simulink model "H175_PANKL_V1a"  (R2023a)
settings: Solver=ode15s  StartTime=0.0  StopTime=22136  RelTol=1e-3  AbsTol=1e-3
PreLoadFcn:
  | omega_TLU = [1000, 1500, 2000, 2500, 3000, 3500];
  | beta_TLU = linspace(0,1,7);
  | 
  | mdot_TLU = [0.1377    0.1304    0.1187    0.1029    0.0854    0.0658    0.0437
  |     0.2310    0.2183    0.1978    0.1688    0.1400    0.1118    0.0750
  |     0.3298    0.3208    0.2987    0.2677    0.2256    0.1774    0.1194
  |     0.4520    0.4260    0.3825    0.3308    0.2745    0.2227    0.1655
  |     0.5542    0.5353    0.4781    0.4230    0.3477    0.2897    0.2211
  |     0.6197    0.5805    0.5198    0.4516    0.3971    0.3555    0.2825];
  | 
  | eta_TLU = [0.7905    0.8025    0.7998    0.7972    0.7932    0.7882    0.7827
  |     0.7993    0.8239    0.8350    0.8379    0.8197    0.8000    0.7809
  |     0.8011    0.8374    0.8632    0.8827    0.8749    0.8394    0.7948
  |     0.8072    0.8520    0.8814    0.9000    0.8676    0.8356    0.7971
  |     0.8076    0.8271    0.8608    0.8766    0.8529    0.8329    0.7992
  |     0.7949    0.8131    0.8296    0.8243    0.8170    0.8085    0.7972];
  | 
  | pr_TLU = [1.0912    1.1795    1.2293    1.2662    1.2928    1.3108    1.3151
  |     1.1484    1.3081    1.3958    1.4707    1.5136    1.5380    1.5456
  |     1.2830    1.4539    1.5943    1.7042    1.7973    1.8582    1.8799
  |     1.5180    1.8034    1.9693    2.0899    2.1662    2.2027    2.2182
  |     1.8359    2.0956    2.3359    2.4668    2.5687    2.6106    2.6224
  |     2.3061    2.6623    2.8585    2.9837    3.0443    3.0714    3.0869];
values from neighbouring files (symbols this model uses):
  P64_omega_TLU = [44762 68636 92509 110414 125335 137271 146224]    [All_Properties.mat]    (also in PANKL_CMP.mat = [44762 68636 92509 110414 125335 137271 146224 155176.0695 1)
libraries: fl_lib x101, nesl_utility x76, SimscapeFluids_lib x5, slpidlib x3
(part 1 of 4)
CloseFcn:
  | clear tout simlogCompressorMap
  | clear omega_TLU
  | clear beta_TLU
  | clear mdot_TLU
  | clear pr_TLU
  | clear eta_TLU
Description:
  | Compressor Map
settings Model: Creator=The MathWorks, Inc.  LastModifiedBy=H2FADMIN
settings SolverCC: AutoScaleAbsTol=off  MaxConsecutiveMinStep=50  ZeroCrossAlgorithm=Adaptive  AlgebraicLoopSolver=TrustRegion  MaxZcPerStep=1
settings DataIOCC: ReturnWorkspaceOutputs=off
settings OptimizationCC: ReuseModelBlockBuffer=off
settings DebuggingCC: AlgebraicLoopMsg=none  IgnoredZcDiagnostic=none  UnconnectedInputMsg=warning  UnconnectedOutputMsg=warning  UnconnectedLineMsg=warning  SymbolicDimsDataTypeCodeGenerationDiagnostic=none
settings ModelReferenceCC: EnableRefExpFcnMdlSchedulingChecks=on
settings SFSimCC: CustomCodeUndefinedFunction=UseInterfaceOnly
settings RTWCC: DLArmComputeVersion=19.05
settings SimscapeCC: SimscapeLogType=all  SimscapeLogSimulationStatistics=on  SimscapeLogName=simlog_H175_PANKL_V1b  SimscapeLogDataHistory=10000

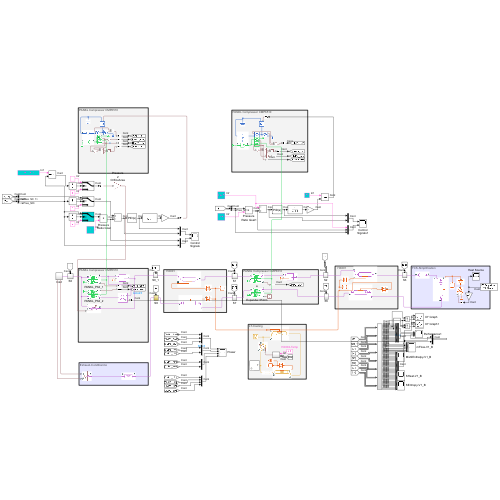
[thumbnail: Simulink's stored preview of the top-level diagram]
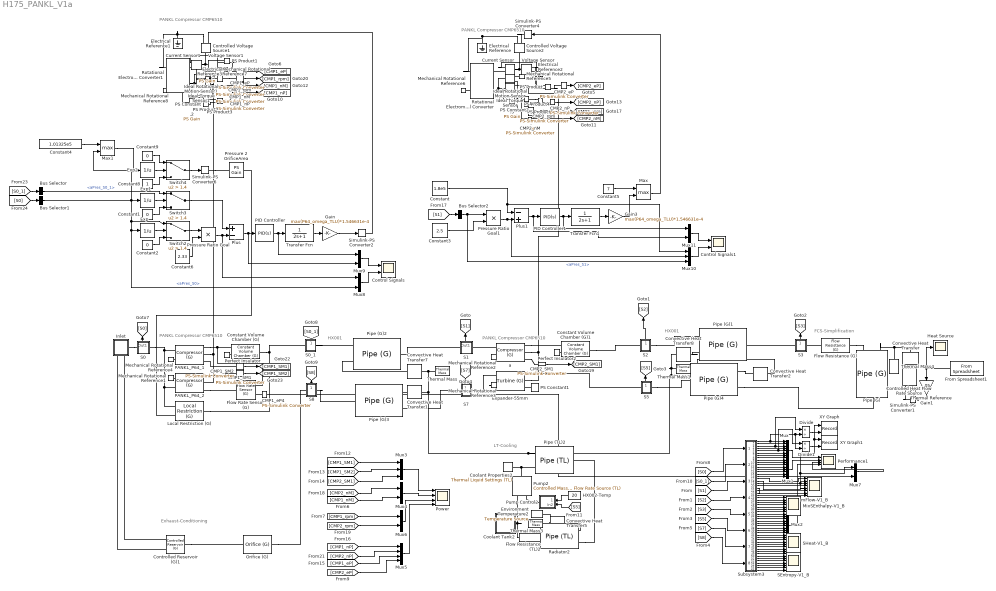
== system H175_PANKL_V1a ==
  note: PANKL Compressor CMP6510
  note: FCS-Simplification
  note: Exhaust-Conditioning
  note: PANKL Compressor CMP6510
  note: HX001
  note: HX001
  note: LT-Cooling
  note: PANKL Compressor CMP6510
  note: PANKL Compressor CMP6510
  . : fl_lib/Physical Signals/Functions/PS Gain  gain=1/(0.1047198*1000)
  .2 : fl_lib/Physical Signals/Functions/PS Gain  gain=1/(0.1047198*60)
  .3 : fl_lib/Physical Signals/Functions/PS Gain  gain=1/(0.1047198*60)
  .4 : fl_lib/Physical Signals/Functions/PS Gain  gain=1/(0.1047198*1000)
  Bus Selector : BusSelector  OutputSignals=aPres_S0_1
  Bus Selector1 : BusSelector  OutputSignals=aPres_S0
  Bus Selector2 : BusSelector  OutputSignals=aPres_S1
  CMP1_SM1 : nesl_utility/PS-Simulink Converter  PhysicalDomain=network_engine_domain  SubClassName=ps_output  LeftPortType=input  RightPortType=output  PseudoPeriodic=off  Frequencies=[]  VectorFormat=inherit  Unit=inherit  AffineConversion=off
  CMP1_SM2 : nesl_utility/PS-Simulink Converter  PhysicalDomain=network_engine_domain  SubClassName=ps_output  LeftPortType=input  RightPortType=output  PseudoPeriodic=off  Frequencies=[]  VectorFormat=inherit  Unit=inherit  AffineConversion=off
  CMP1_eP : nesl_utility/PS-Simulink Converter  PhysicalDomain=network_engine_domain  SubClassName=ps_output  LeftPortType=input  RightPortType=output  PseudoPeriodic=off  Frequencies=[]  VectorFormat=inherit  Unit=inherit  AffineConversion=off
  CMP1_eP4 : nesl_utility/PS-Simulink Converter  PhysicalDomain=network_engine_domain  SubClassName=ps_output  LeftPortType=input  RightPortType=output  PseudoPeriodic=off  Frequencies=[]  VectorFormat=inherit  Unit=inherit  AffineConversion=off
  CMP1_nM : nesl_utility/PS-Simulink Converter  PhysicalDomain=network_engine_domain  SubClassName=ps_output  LeftPortType=input  RightPortType=output  PseudoPeriodic=off  Frequencies=[]  VectorFormat=1-D array  Unit=inherit  AffineConversion=off
  CMP1_nP : nesl_utility/PS-Simulink Converter  PhysicalDomain=network_engine_domain  SubClassName=ps_output  LeftPortType=input  RightPortType=output  PseudoPeriodic=off  Frequencies=[]  VectorFormat=inherit  Unit=inherit  AffineConversion=off
  CMP1_rpm : nesl_utility/PS-Simulink Converter  PhysicalDomain=network_engine_domain  SubClassName=ps_output  LeftPortType=input  RightPortType=output  PseudoPeriodic=off  Frequencies=[]  VectorFormat=inherit  Unit=inherit  AffineConversion=off
  CMP2_SM1 : nesl_utility/PS-Simulink Converter  PhysicalDomain=network_engine_domain  SubClassName=ps_output  LeftPortType=input  RightPortType=output  PseudoPeriodic=off  Frequencies=[]  VectorFormat=inherit  Unit=inherit  AffineConversion=off
  CMP2_eP : nesl_utility/PS-Simulink Converter  PhysicalDomain=network_engine_domain  SubClassName=ps_output  LeftPortType=input  RightPortType=output  PseudoPeriodic=off  Frequencies=[]  VectorFormat=inherit  Unit=inherit  AffineConversion=off
  CMP2_nM : nesl_utility/PS-Simulink Converter  PhysicalDomain=network_engine_domain  SubClassName=ps_output  LeftPortType=input  RightPortType=output  PseudoPeriodic=off  Frequencies=[]  VectorFormat=1-D array  Unit=inherit  AffineConversion=off
  CMP2_nP : nesl_utility/PS-Simulink Converter  PhysicalDomain=network_engine_domain  SubClassName=ps_output  LeftPortType=input  RightPortType=output  PseudoPeriodic=off  Frequencies=[]  VectorFormat=inherit  Unit=inherit  AffineConversion=off
  CMP2_rpm : nesl_utility/PS-Simulink Converter  PhysicalDomain=network_engine_domain  SubClassName=ps_output  LeftPortType=input  RightPortType=output  PseudoPeriodic=off  Frequencies=[]  VectorFormat=inherit  Unit=inherit  AffineConversion=off
  Constant : Constant  Value=1.8e5
  Constant Volume Chamber (G) : fl_lib/Gas/Elements/Constant Volume Chamber (G)  volume=1 l  num_ports=foundation.enum.num_ports.two  area_A=0.1 m^2  area_B=0.005 m^2  area_C=0.01 m^2  area_D=0.01 m^2  p_I_specify=off  p_I_priority=High  p_I=0.101325 MPa  p_I_nominal_specify=off  p_I_nominal_unit=MPa  p_I_nominal_value=1  T_I_specify=off  T_I_priority=High  T_I=293.15 K  T_I_nominal_specify=off  T_I_nominal_unit=K  T_I_nominal_value=1  rho_I_specify=off  rho_I_priority=None  rho_I=1.2 kg/m^3  rho_I_nominal_specify=off  rho_I_nominal_unit=kg/m^3  rho_I_nominal_value=1
      settings: InternalSimscapePortConfiguration="{\"Bottom\":[],\"Left\":[{\"id\":\"A\",\"label\":\"A\",\"type\":\"foundation.gas.gas\"},{\"id\":\"H\",\"label\":\"H\",\"type\":\"foundation.thermal.thermal\"}],\"Right\":[{\"id\":\"B\",\"label\":\"B\",\"type\":\"foundation.gas.gas\"}],\"Top\":[]}"
  Constant Volume Chamber (G)1 : fl_lib/Gas/Elements/Constant Volume Chamber (G)  volume=1 l  num_ports=foundation.enum.num_ports.two  area_A=0.1 m^2  area_B=0.005 m^2  area_C=0.01 m^2  area_D=0.01 m^2  p_I_specify=off  p_I_priority=High  p_I=0.101325 MPa  p_I_nominal_specify=off  p_I_nominal_unit=MPa  p_I_nominal_value=1  T_I_specify=off  T_I_priority=High  T_I=293.15 K  T_I_nominal_specify=off  T_I_nominal_unit=K  T_I_nominal_value=1  rho_I_specify=off  rho_I_priority=None  rho_I=1.2 kg/m^3  rho_I_nominal_specify=off  rho_I_nominal_unit=kg/m^3  rho_I_nominal_value=1
      settings: InternalSimscapePortConfiguration="{\"Bottom\":[],\"Left\":[{\"id\":\"A\",\"label\":\"A\",\"type\":\"foundation.gas.gas\"},{\"id\":\"H\",\"label\":\"H\",\"type\":\"foundation.thermal.thermal\"}],\"Right\":[{\"id\":\"B\",\"label\":\"B\",\"type\":\"foundation.gas.gas\"}],\"Top\":[]}"
  Constant1 : Constant  Value=0
  Constant2 : Constant  Value=0
  Constant3 : Constant  Value=2.5
  Constant4 : Constant  Value=1.01325e5
  Constant5 : Constant  Value=7
  Constant6 : Constant  Value=2.33
  Constant8 : Constant
  Constant9 : Constant  Value=0
  Control Signals : Scope  NumInputPorts=2
  Control Signals1 : Scope  NumInputPorts=2
  Controlled Heat Flow Rate Source : fl_lib/Thermal/Thermal Sources/Controlled Heat Flow Rate Source
  Controlled Reservoir (G)1 : fl_lib/Gas/Elements/Controlled Reservoir (G)  area_A=0.002 m^2
      settings: InternalSimscapePortConfiguration="{\"Bottom\":[],\"Left\":[{\"id\":\"A\",\"label\":\"A\",\"type\":\"foundation.gas.gas\"}],\"Right\":[{\"id\":\"T_in\",\"label\":\"T\",\"type\":\"input\"},{\"id\":\"p_in\",\"label\":\"P\",\"type\":\"input\"}],\"Top\":[]}"
  Controlled Voltage Source1 : fl_lib/Electrical/Electrical Sources/Controlled Voltage Source
  Controlled Voltage Source2 : fl_lib/Electrical/Electrical Sources/Controlled Voltage Source
  Convective Heat Transfer : fl_lib/Thermal/Thermal Elements/Convective Heat Transfer  thermal_type=foundation.enum.constant_variable.constant  area=.25 m^2  heat_tr_coeff=200 W/(K*m^2)  min_heat_tr_coeff=1e-3 W/(K*m^2)  T_specify=on  T_priority=None  T=10 K  T_nominal_specify=off  T_nominal_unit=K  T_nominal_value=1  Q_specify=off  Q_priority=None  Q=0 W  Q_nominal_specify=off  Q_nominal_unit=W  Q_nominal_value=1
  Convective Heat Transfer1 : fl_lib/Thermal/Thermal Elements/Convective Heat Transfer  thermal_type=foundation.enum.constant_variable.constant  area=100 cm^2  heat_tr_coeff=1000 W/(m^2 * K)  min_heat_tr_coeff=1e-3 W/(K*m^2)  T_specify=off  T_priority=None  T=0 K  T_nominal_specify=off  T_nominal_unit=K  T_nominal_value=1  Q_specify=off  Q_priority=None  Q=0 W  Q_nominal_specify=off  Q_nominal_unit=W  Q_nominal_value=1
  Convective Heat Transfer2 : fl_lib/Thermal/Thermal Elements/Convective Heat Transfer  thermal_type=foundation.enum.constant_variable.constant  area=100 cm^2  heat_tr_coeff=1000 W/(m^2 * K)  min_heat_tr_coeff=1e-3 W/(K*m^2)  T_specify=off  T_priority=None  T=0 K  T_nominal_specify=off  T_nominal_unit=K  T_nominal_value=1  Q_specify=off  Q_priority=None  Q=0 W  Q_nominal_specify=off  Q_nominal_unit=W  Q_nominal_value=1
  Convective Heat Transfer5 : fl_lib/Thermal/Thermal Elements/Convective Heat Transfer  thermal_type=foundation.enum.constant_variable.constant  area=5 m^2  heat_tr_coeff=300 W/(m^2 * K)  min_heat_tr_coeff=1e-3 W/(K*m^2)  T_specify=off  T_priority=None  T=0 K  T_nominal_specify=off  T_nominal_unit=K  T_nominal_value=1  Q_specify=off  Q_priority=None  Q=0 W  Q_nominal_specify=off  Q_nominal_unit=W  Q_nominal_value=1
  Convective Heat Transfer7 : fl_lib/Thermal/Thermal Elements/Convective Heat Transfer  thermal_type=foundation.enum.constant_variable.constant  area=100 cm^2  heat_tr_coeff=50000 W/(m^2 * K)  min_heat_tr_coeff=1e-3 W/(K*m^2)  T_specify=off  T_priority=None  T=0 K  T_nominal_specify=off  T_nominal_unit=K  T_nominal_value=1  Q_specify=off  Q_priority=None  Q=0 W  Q_nominal_specify=off  Q_nominal_unit=W  Q_nominal_value=1
  Convective Heat Transfer8 : fl_lib/Thermal/Thermal Elements/Convective Heat Transfer  thermal_type=foundation.enum.constant_variable.constant  area=100 cm^2  heat_tr_coeff=100000 W/(m^2 * K)  min_heat_tr_coeff=1e-3 W/(K*m^2)  T_specify=off  T_priority=None  T=0 K  T_nominal_specify=off  T_nominal_unit=K  T_nominal_value=1  Q_specify=off  Q_priority=None  Q=0 W  Q_nominal_specify=off  Q_nominal_unit=W  Q_nominal_value=1
  Coolant Properties2 : fl_lib/Thermal Liquid/Utilities/Thermal Liquid Settings (TL)  table_dimensions=foundation.enum.table_dimensions_TL.two_dimensional  T_TLU=[273.1600 : 10 : 373.16]' K  p_TLU=[0.01, 0.1, 5 : 5 : 50] MPa  p_atm=0.101325 MPa  pT_region_flag=foundation.enum.pT_region_TL.min_max  T_min=273.16 K  T_max=373.16 K  p_min=0.05 MPa  p_max=50 MPa  T_min_1D=273.16 K  T_max_1D=363.16 K  p_min_1D=0.05 MPa  p_max_1D=50 MPa  pT_validity_TLU=[1, 1, 1, 1, 1, 1, 1, 1, 1, 1, 1, 1; 1, 1, 1, 1, 1, 1, 1, 1, 1, 1, 1, 1; 1, 1, 1, 1, 1, 1, 1, 1, 1, 1, 1, 1; 1, 1, 1, 1, 1, 1, 1, 1, 1, 1, 1, 1; 1, 1, 1, 1, 1, 1, 1, 1, 1, 1, 1, 1; 0, 1, 1, 1, 1, 1, 1, 1, 1, 1, 1, 1; 0, 1, 1, 1, 1, 1, 1, 1, 1, 1, 1, 1; 0, 1, 1, 1, 1, 1, 1, 1, 1, 1, 1, 1; 0, 1, 1, 1, 1, 1, 1, 1, 1, 1, 1, 1; 0, 1, 1, 1, 1, 1, 1, 1, 1, 1, 1, 1; 0, 0, 1, 1, 1, 1, 1, 1, 1, 1, 1, 1]  properties_range_check=simscape.enum.assert.action.error  rho_parameterization_2D=foundation.enum.rho_parameterization_2D.rho_beta_alpha  rho_parameterization_1D=foundation.enum.rho_parameterization_1D.rho_vector  rho_TLU=[999.7973, 999.8431, 1002.3216, 1004.8218, 1007.293, 1009.7358, 1012.1506, 1014.5379, 1016.8979, 1019.2311, 1021.538, 1023.8188; 999.6579, 999.7009, 1002.0303, 1004.382, 1006.7084, 1009.0101, 1011.2874, 1013.5407, 1015.7703, 1017.9766, 1020.1599, 1022.3206; 998.1632, 998.2045, 1000.4375, 1002.6924, 1004.9239, 1007.1324, 1009.3183, 1011.4819, 1013.6236, 1015.7438, 1017.8428, 1019.921; 995.6057, 995.6458, 997.81864, 1000.0128, 1002.1841, 1004.3332, 1006.4603, 1008.566, 1010.6505, 1012.7144, 1014.758, 1016.7815; 992.1724, 992.2119, 994.35133, 996.5113, 998.6484, 1000.7633, 1002.8563, 1004.928, 1006.9788, 1009.009, 1011.0192, 1013.0097; 988.02, 988.0299, 990.15684, 992.3035, 994.4268, 996.5273, 998.6056, 1000.6622, 1002.6976, 1004.7123, 1006.7067, 1008.6813; 983.18, 983.1901, 985.3217, 987.4721, 989.5983, 991.7008, 993.7803, 995.8374, 997.8726, 999.8864, 1001.8795, 1003.8522; 977.75, 977.7583, 979.9094, 982.0783, 984.2216, 986.34, 988.4343, 990.505, 992.5529, 994.5786, 996.5825, 998.5654; 971.77, 971.7836, 973.96734, 976.1678, 978.3409, 980.4876, 982.6087, 984.7049, 986.7768, 988.8254, 990.8511, 992.8545; 965.26, 965.3023, 967.53107, 969.7753, 971.9901, 974.1764, 976.3354, 978.4676, 980.5741, 982.6556, 984.7129, 986.7465; 958.62, 958.6315, 960.627, 962.9267, 965.1944, 967.4314, 969.6387, 971.8173, 973.9681, 976.0921, 978.19, 980.2628] kg/m^3  beta_TLU=[1.9649, 1.9654, 1.9929, 2.0213, 2.0499, 2.0787, 2.1078, 2.1372, 2.1668, 2.1966, 2.2268, 2.2572; 2.0913, 2.0918, 2.1191, 2.1471, 2.1752, 2.2036, 2.2322, 2.261, 2.2899, 2.3191, 2.3485, 2.3781; 2.1786, 2.1791, 2.2067, 2.235, 2.2634, 2.2919, 2.3206, 2.3494, 2.3784, 2.4075, 2.4367, 2.4661; 2.2332, 2.2337, 2.2619, 2.2908, 2.3197, 2.3487, 2.3778, 2.407, 2.4363, 2.4657, 2.4951, 2.5246; 2.26, 2.2605, 2.2895, 2.3191, 2.3487, 2.3784, 2.4081, 2.4378, 2.4675, 2.4973, 2.5272, 2.5571; 2.2638, 2.2638, 2.2936, 2.324, 2.3544, 2.3848, 2.4151, 2.4455, 2.4758, 2.5062, 2.5365, 2.5669; 2.2472, 2.2472, 2.2779, 2.3092, 2.3403, 2.3715, 2.4025, 2.4336, 2.4646, 2.4955, 2.5264, 2.5573; 2.214, 2.214, 2.2455, 2.2776, 2.3096, 2.3415, 2.3733, 2.405, 2.4367, 2.4683, 2.4998, 2.5313; 2.1668, 2.1668, 2.1992, 2.2321, 2.2649, 2.2976, 2.3301, 2.3626, 2.3949, 2.4272, 2.4593, 2.4914; 2.1081, 2.1081, 2.1413, 2.175, 2.2086, 2.2421, 2.2754, 2.3085, 2.3415, 2.3744, 2.4072, 2.4399; 2.0494, 2.0494, 2.0739, 2.1084, 2.1428, 2.177, 2.211, 2.2449, 2.2786, 2.3121, 2.3455, 2.3788] GPa  alpha_TLU=1e-4 * [-.679, -.676, -.49, -.307, -.13, .041, .206, .365, .519, .668, .811, .949; .878, .881, .998, 1.114, 1.227, 1.337, 1.445, 1.549, 1.651, 1.75, 1.846, 1.939; 2.068, 2.069, 2.141, 2.213, 2.283, 2.352, 2.42, 2.486, 2.551, 2.614, 2.676, 2.736; 3.034, 3.035, 3.074, 3.113, 3.152, 3.191, 3.229, 3.267, 3.305, 3.341, 3.377, 3.413; 3.855, 3.856, 3.87, 3.884, 3.899, 3.914, 3.93, 3.946, 3.961, 3.977, 3.993, 4.009; 4.578, 4.578, 4.572, 4.566, 4.562, 4.558, 4.555, 4.552, 4.55, 4.549, 4.548, 4.547; 5.233, 5.233, 5.209, 5.186, 5.165, 5.144, 5.125, 5.107, 5.09, 5.074, 5.059, 5.045; 5.84, 5.84, 5.801, 5.762, 5.725, 5.691, 5.657, 5.625, 5.595, 5.566, 5.538, 5.512; 6.414, 6.414, 6.36, 6.307, 6.256, 6.208, 6.161, 6.117, 6.074, 6.033, 5.994, 5.956; 6.967, 6.967, 6.898, 6.831, 6.766, 6.705, 6.646, 6.589, 6.535, 6.482, 6.432, 6.384; 7.519, 7.519, 7.423, 7.342, 7.264, 7.189, 7.118, 7.049, 6.983, 6.92, 6.859, 6.8] 1/K  rho_TLU_2=[999.7973, 999.8431, 1002.3216, 1004.8218, 1007.293, 1009.7358, 1012.1506, 1014.5379, 1016.8979, 1019.2311, 1021.538, 1023.8188; 999.6579, 999.7009, 1002.0303, 1004.382, 1006.7084, 1009.0101, 1011.2874, 1013.5407, 1015.7703, 1017.9766, 1020.1599, 1022.3206; 998.1632, 998.2045, 1000.4375, 1002.6924, 1004.9239, 1007.1324, 1009.3183, 1011.4819, 1013.6236, 1015.7438, 1017.8428, 1019.921; 995.6057, 995.6458, 997.81864, 1000.0128, 1002.1841, 1004.3332, 1006.4603, 1008.566, 1010.6505, 1012.7144, 1014.758, 1016.7815; 992.1724, 992.2119, 994.35133, 996.5113, 998.6484, 1000.7633, 1002.8563, 1004.928, 1006.9788, 1009.009, 1011.0192, 1013.0097; 988.02, 988.0299, 990.15684, 992.3035, 994.4268, 996.5273, 998.6056, 1000.6622, 1002.6976, 1004.7123, 1006.7067, 1008.6813; 983.18, 983.1901, 985.3217, 987.4721, 989.5983, 991.7008, 993.7803, 995.8374, 997.8726, 999.8864, 1001.8795, 1003.8522; 977.75, 977.7583, 979.9094, 982.0783, 984.2216, 986.34, 988.4343, 990.505, 992.5529, 994.5786, 996.5825, 998.5654; 971.77, 971.7836, 973.96734, 976.1678, 978.3409, 980.4876, 982.6087, 984.7049, 986.7768, 988.8254, 990.8511, 992.8545; 965.26, 965.3023, 967.53107, 969.7753, 971.9901, 974.1764, 976.3354, 978.4676, 980.5741, 982.6556, 984.7129, 986.7465; 958.62, 958.6315, 960.627, 962.9267, 965.1944, 967.4314, 969.6387, 971.8173, 973.9681, 976.0921, 978.19, 980.2628] kg/m^3  rho_ref_3=998.21 kg/m^3  T_ref_3=293.16 K  p_ref_3=0.101325 MPa  beta_const_3=2.1791 GPa  alpha_const_3=2.0691e-4 1/K  rho_TLU_4=[999.84; 999.7; 998.2; 995.65; 992.21; 988.03; 983.19; 977.76; 971.78; 965.3; 958.8] kg/m^3  beta_const_4=2.1791 GPa  p_ref_4=0.101325 MPa  rho_ref_5=998.21 kg/m^3  T_ref_5=293.16 K  p_ref_5=0.101325 MPa  beta_const_5=2.1791 GPa  alpha_const_5=2.0691e-4 1/K  u_parameterization_2D=foundation.enum.u_parameterization_2D.u_cp  u_parameterization_1D=foundation.enum.u_parameterization_1D.u  u_TLU=[.0002, .0018, .086, .1588, .219, .267, .3034, .3288, .3436, .3483, .3435, .3294; 42.062, 42.06, 41.935, 41.804, 41.668, 41.527, 41.382, 41.233, 41.081, 40.924, 40.763, 40.599; 83.953, 83.948, 83.651, 83.349, 83.049, 82.749, 82.451, 82.153, 81.856, 81.56, 81.265, 80.971; 125.77, 125.76, 125.31, 124.86, 124.41, 123.97, 123.53, 123.1, 122.68, 122.25, 121.84, 121.42; 167.57, 167.56, 166.96, 166.37, 165.79, 165.21, 164.65, 164.09, 163.54, 163, 162.46, 161.94; 209.36, 209.36, 208.63, 207.9, 207.19, 206.48, 205.79, 205.11, 204.45, 203.79, 203.14, 202.5; 251.19, 251.19, 250.33, 249.47, 248.62, 247.79, 246.98, 246.18, 245.39, 244.62, 243.86, 243.12; 293.06, 293.06, 292.07, 291.07, 290.1, 289.14, 288.2, 287.28, 286.38, 285.49, 284.62, 283.77; 334.99, 334.99, 333.86, 332.73, 331.63, 330.54, 329.48, 328.44, 327.41, 326.41, 325.43, 324.46; 377, 377, 375.73, 374.46, 373.22, 372, 370.81, 369.64, 368.5, 367.38, 366.27, 365.19; 419.01, 419.01, 417.69, 416.27, 414.89, 413.54, 412.21, 410.91, 409.64, 408.4, 407.17, 405.98] kJ/kg  cp_TLU=[4.2199, 4.2194, 4.1957, 4.1726, 4.1508, 4.13, 4.1103, 4.0916, 4.0738, 4.0569, 4.0408, 4.0254; 4.1955, 4.1951, 4.1769, 4.1592, 4.1422, 4.1259, 4.1103, 4.0954, 4.0812, 4.0676, 4.0545, 4.0421; 4.1843, 4.184, 4.169, 4.1543, 4.1401, 4.1264, 4.1133, 4.1007, 4.0885, 4.0768, 4.0656, 4.0548; 4.1801, 4.1798, 4.1667, 4.1538, 4.1413, 4.1293, 4.1177, 4.1064, 4.0956, 4.0851, 4.075, 4.0653; 4.1796, 4.1794, 4.1675, 4.1558, 4.1444, 4.1334, 4.1227, 4.1123, 4.1023, 4.0926, 4.0832, 4.0741; 4.1813, 4.1813, 4.1702, 4.1592, 4.1484, 4.138, 4.1279, 4.1181, 4.1086, 4.0993, 4.0903, 4.0816; 4.185, 4.185, 4.1742, 4.1636, 4.1532, 4.1432, 4.1334, 4.1239, 4.1146, 4.1056, 4.0969, 4.0884; 4.1901, 4.1901, 4.1795, 4.169, 4.1588, 4.1489, 4.1393, 4.1299, 4.1207, 4.1118, 4.1032, 4.0947; 4.1968, 4.1968, 4.1862, 4.1757, 4.1655, 4.1555, 4.1458, 4.1364, 4.1273, 4.1183, 4.1096, 4.1012; 4.2052, 4.2052, 4.1944, 4.1837, 4.1733, 4.1632, 4.1534, 4.1438, 4.1345, 4.1255, 4.1166, 4.108; 4.2136, 4.2136, 4.2045, 4.1935, 4.1828, 4.1724, 4.1623, 4.1524, 4.1429, 4.1335, 4.1245, 4.1157] kJ/kg/K  u_TLU_2=[.0002, .0018, .086, .1588, .219, .267, .3034, .3288, .3436, .3483, .3435, .3294; 42.062, 42.06, 41.935, 41.804, 41.668, 41.527, 41.382, 41.233, 41.081, 40.924, 40.763, 40.599; 83.953, 83.948, 83.651, 83.349, 83.049, 82.749, 82.451, 82.153, 81.856, 81.56, 81.265, 80.971; 125.77, 125.76, 125.31, 124.86, 124.41, 123.97, 123.53, 123.1, 122.68, 122.25, 121.84, 121.42; 167.57, 167.56, 166.96, 166.37, 165.79, 165.21, 164.65, 164.09, 163.54, 163, 162.46, 161.94; 209.36, 209.36, 208.63, 207.9, 207.19, 206.48, 205.79, 205.11, 204.45, 203.79, 203.14, 202.5; 251.19, 251.19, 250.33, 249.47, 248.62, 247.79, 246.98, 246.18, 245.39, 244.62, 243.86, 243.12; 293.06, 293.06, 292.07, 291.07, 290.1, 289.14, 288.2, 287.28, 286.38, 285.49, 284.62, 283.77; 334.99, 334.99, 333.86, 332.73, 331.63, 330.54, 329.48, 328.44, 327.41, 326.41, 325.43, 324.46; 377, 377, 375.73, 374.46, 373.22, 372, 370.81, 369.64, 368.5, 367.38, 366.27, 365.19; 419.01, 419.01, 417.69, 416.27, 414.89, 413.54, 412.21, 410.91, 409.64, 408.4, 407.17, 405.98] kJ/kg  cp_TLU_3=[4.2199, 4.2194, 4.1957, 4.1726, 4.1508, 4.13, 4.1103, 4.0916, 4.0738, 4.0569, 4.0408, 4.0254; 4.1955, 4.1951, 4.1769, 4.1592, 4.1422, 4.1259, 4.1103, 4.0954, 4.0812, 4.0676, 4.0545, 4.0421; 4.1843, 4.184, 4.169, 4.1543, 4.1401, 4.1264, 4.1133, 4.1007, 4.0885, 4.0768, 4.0656, 4.0548; 4.1801, 4.1798, 4.1667, 4.1538, 4.1413, 4.1293, 4.1177, 4.1064, 4.0956, 4.0851, 4.075, 4.0653; 4.1796, 4.1794, 4.1675, 4.1558, 4.1444, 4.1334, 4.1227, 4.1123, 4.1023, 4.0926, 4.0832, 4.0741; 4.1813, 4.1813, 4.1702, 4.1592, 4.1484, 4.138, 4.1279, 4.1181, 4.1086, 4.0993, 4.0903, 4.0816; 4.185, 4.185, 4.1742, 4.1636, 4.1532, 4.1432, 4.1334, 4.1239, 4.1146, 4.1056, 4.0969, 4.0884; 4.1901, 4.1901, 4.1795, 4.169, 4.1588, 4.1489, 4.1393, 4.1299, 4.1207, 4.1118, 4.1032, 4.0947; 4.1968, 4.1968, 4.1862, 4.1757, 4.1655, 4.1555, 4.1458, 4.1364, 4.1273, 4.1183, 4.1096, 4.1012; 4.2052, 4.2052, 4.1944, 4.1837, 4.1733, 4.1632, 4.1534, 4.1438, 4.1345, 4.1255, 4.1166, 4.108; 4.2136, 4.2136, 4.2045, 4.1935, 4.1828, 4.1724, 4.1623, 4.1524, 4.1429, 4.1335, 4.1245, 4.1157] kJ/kg/K  u_TLU_4=[.0018; 42.06; 83.948; 125.76; 167.56; 209.36; 251.19; 293.06; 334.99; 377; 418.01] kJ/kg  cp_TLU_5=[4.2199; 4.1955; 4.1843; 4.1801; 4.1796; 4.1813; 4.185; 4.1901; 4.1968; 4.2052; 4.2136] kJ/kg/K  nu_TLU=[1.7917, 1.7914, 1.7763, 1.7615, 1.7473, 1.7338, 1.7208, 1.7085, 1.6967, 1.6854, 1.6747, 1.6645; 1.3061, 1.3059, 1.2986, 1.2914, 1.2845, 1.2779, 1.2716, 1.2656, 1.2598, 1.2543, 1.2491, 1.2441; 1.0032, 1.0032, .9995, .9959, .9924, .9891, .9859, .9829, .9801, .9774, .9748, .9724; .8006, .8005, .7987, .797, .7953, .7937, .7922, .7908, .7894, .7881, .787, .7859; .6577, .6577, .657, .6562, .6555, .6548, .6543, .6537, .6532, .6528, .6523, .652; .553, .553, .5529, .5527, .5526, .5525, .5524, .5524, .5524, .5524, .5524, .5525; .4739, .4739, .4741, .4743, .4745, .4747, .475, .4753, .4755, .4758, .4762, .4765; .4127, .4127, .4131, .4135, .4139, .4143, .4148, .4152, .4157, .4162, .4167, .4172; .3643, .3643, .3648, .3654, .3659, .3665, .367, .3676, .3682, .3688, .3694, .37; .3254, .3254, .3261, .3267, .3273, .328, .3286, .3293, .3299, .3306, .3312, .3319; .2866, .2866, .2945, .2952, .2959, .2965, .2972, .2979, .2986, .2993, .3, .3007] mm^2/s  nu_TLU_2=[1.7917; 1.3061; 1.0032; .8006; .6577; .553; .4739; .4127; .3643; .3254; .2866] mm^2/s  k_TLU=[561.04, 561.09, 563.8, 566.56, 569.32, 572.08, 574.82, 577.54, 580.24, 582.92, 585.57, 588.18; 580.02, 580.07, 582.45, 584.88, 587.32, 589.75, 592.18, 594.61, 597.02, 599.42, 601.8, 604.16; 598.44, 598.48, 600.73, 603.03, 605.33, 607.64, 609.94, 612.24, 614.54, 616.82, 619.1, 621.36; 615.48, 615.52, 617.73, 620, 622.26, 624.54, 626.81, 629.07, 631.34, 633.6, 635.85, 638.09; 630.6, 630.64, 632.87, 635.15, 637.44, 639.72, 642.01, 644.29, 646.57, 648.84, 651.11, 653.36; 643.61, 643.61, 645.88, 648.21, 650.53, 652.86, 655.18, 657.51, 659.82, 662.14, 664.44, 666.74; 654.39, 654.39, 656.73, 659.12, 661.5, 663.89, 666.27, 668.65, 671.02, 673.38, 675.74, 678.09; 663.13, 663.13, 665.54, 668, 670.46, 672.91, 675.36, 677.8, 680.24, 682.67, 685.09, 687.5; 670.02, 670.02, 672.51, 675.05, 677.59, 680.12, 682.64, 685.16, 687.67, 690.17, 692.66, 695.14; 675.27, 675.27, 677.85, 680.48, 683.11, 685.73, 688.34, 690.94, 693.53, 696.11, 698.68, 701.24; 680.52, 680.52, 681.77, 684.5, 687.22, 689.94, 692.64, 695.34, 698.02, 700.69, 703.35, 706] mW/m/K  k_TLU_2=[561.04; 580.02; 598.44; 615.48; 630.6; 643.61; 654.39; 663.13; 670.02; 675.27; 680.52] mW/m/K
  Coolant Tank2 : Subsystem  Tag=PublishSubsystem  mask(Coolant Tank){A=1, x_init=0.08}
      mask prompts: A "Tank area (m^2)"; x_init "Initial coolant level (m)"
      mask help: This subsystem models an expansion tank for the coolant system.
  Current Sensor : fl_lib/Electrical/Electrical Sensors/Current Sensor
  Current Sensor1 : fl_lib/Electrical/Electrical Sensors/Current Sensor
  Divide : Product  Inputs=*/
  Divide1 : Product  Inputs=*/
  Electrical Reference{,1..3} (4 alike) : fl_lib/Electrical/Electrical Elements/Electrical Reference
  Environment Temperature2 : fl_lib/Thermal/Thermal Sources/Temperature Source  temperature=20 degC
  Exp : Math  Operator=reciprocal
  Exp1 : Math  Operator=reciprocal
  Exp2 : Math  Operator=reciprocal
  Expander-55mm : SimscapeFluids_lib/Gas/Turbomachinery/Turbine (G)  parameterization=fluids.gas.turbomachinery.enum.TurbineParameterization.Tabulated1D  omega_TLU_2=[31000, 45000, 60000, 75000, 90000, 105000, 120000] rpm  variable_nozzle=true  min_nozzle_opening=1e-3  max_nozzle_opening=1  pr_nom=2  mdot_nom=0.08 kg/s  pr_mdot_TLU=[1.0400, 1.0600, 1.1000, 1.1500, 1.2400, 1.3000, 1.3700, 1.5000, 1.6600, 1.7700, 1.8200, 1.9000]  mdot_TLU=[0.0535, 0.0705, 0.0923, 0.1170, 0.1467, 0.1675, 0.1802, 0.2004, 0.2171, 0.2375, 0.2454, 0.25702] kg/s  pr_mdot_TLU_2=[1.217, 1.285, 1.323, 1.363, 1.402, 1.427, 1.495, 1.545, 1.6, 1.687, 1.747, 1.8074; 1.231, 1.302, 1.356, 1.404, 1.443, 1.473, 1.525, 1.577, 1.635, 1.709, 1.782, 1.845; 1.242, 1.328, 1.388, 1.437, 1.528, 1.617, 1.704, 1.811, 1.915, 1.979, 2.053, 2.1226; 1.244, 1.339, 1.417, 1.465, 1.528, 1.584, 1.692, 1.787, 1.899, 2, 2.075, 2.1492; 1.245, 1.34, 1.425, 1.492, 1.546, 1.684, 1.748, 1.882, 1.987, 2.084, 2.167, 2.2458; 1.251, 1.345, 1.442, 1.521, 1.596, 1.692, 1.849, 1.972, 2.1, 2.173, 2.259, 2.3424; 1.248, 1.348, 1.447, 1.516, 1.581, 1.651, 1.749, 1.839, 1.93, 2.024, 2.154, 2.242]  mdot_TLU_2=[40.403, 44.417, 46.653, 47.966, 48.97, 49.544, 50.001, 50.081, 50.086, 50.095, 50.09, 50.0922; 40.044, 43.754, 46.125, 47.626, 48.513, 49.105, 49.481, 49.58, 49.597, 49.624, 49.638, 49.633; 39.941, 43.795, 46.017, 47.335, 48.795, 49.199, 49.279, 49.27, 49.248, 49.23, 49.255, 49.2428; 39.896, 43.512, 45.914, 47.061, 48.011, 48.558, 48.943, 49.042, 49.069, 49.01, 49.046, 49.0266; 39.524, 42.934, 45.686, 46.743, 47.715, 48.67, 48.777, 48.836, 48.876, 48.836, 48.845, 48.8184; 39.439, 43.01, 45.556, 46.801, 47.792, 48.388, 48.634, 48.67, 48.639, 48.647, 48.625, 48.5912; 39.502, 42.849, 45.336, 46.385, 47.312, 47.877, 48.222, 48.397, 48.459, 48.482, 48.455, 48.414] kg/s  efficiency_constant=.954  pr_eta_TLU=[1.0300, 1.0400, 1.0500, 1.1000, 1.1800, 1.2500, 1.3000, 1.4200, 1.5100, 1.6500, 1.7200, 1.8200]  eta_TLU=[0.6590, 0.7100, 0.7730, 0.7910, 0.8180, 0.8850, 0.9190, 0.9450, 0.9280, 0.9090, 0.8840, 0.8210]  pr_eta_TLU_2=[1.224, 1.246, 1.292, 1.387, 1.457, 1.534, 1.61, 1.686, 1.743, 1.79, 1.871, 1.914; 1.237, 1.25, 1.28, 1.369, 1.459, 1.553, 1.629, 1.716, 1.799, 1.846, 1.927, 1.97; 1.241, 1.255, 1.283, 1.326, 1.401, 1.509, 1.591, 1.704, 1.806, 1.913, 1.994, 2.037; 1.25, 1.265, 1.308, 1.364, 1.456, 1.532, 1.637, 1.739, 1.851, 1.934, 2.042, 2.085; 1.281, 1.314, 1.371, 1.425, 1.498, 1.574, 1.647, 1.749, 1.878, 1.979, 2.091, 2.18; 1.252, 1.328, 1.425, 1.544, 1.642, 1.757, 1.873, 2.005, 2.1, 2.204, 2.248, 2.28; 1.382, 1.43, 1.495, 1.586, 1.688, 1.791, 1.887, 1.99, 2.079, 2.158, 2.249, 2.36]  eta_TLU_2=[.72, .754, .759, .739, .714, .679, .643, .603, .554, .524, .494, .48; .716, .757, .794, .819, .812, .788, .761, .728, .692, .662, .632, .618; .629, .691, .775, .831, .858, .869, .859, .842, .816, .782, .752, .738; .594, .668, .757, .804, .857, .883, .892, .893, .884, .865, .835, .821; .664, .72, .779, .823, .858, .883, .897, .905, .904, .896, .883, .868; .559, .61, .673, .741, .788, .835, .869, .895, .908, .899, .854, .751; .718, .785, .824, .855, .882, .9, .908, .906, .884, .857, .804, .701]  p_reference=0.101325 MPa  T_reference=293 K  mechanical_efficiency=0.9  area_A=0.002 m^2  area_B=0.002 m^2
      settings: InternalSimscapePortConfiguration="{\"Bottom\":[],\"Left\":[{\"id\":\"A\",\"label\":\"A\",\"type\":\"foundation.gas.gas\"},{\"id\":\"R\",\"label\":\"R\",\"type\":\"foundation.mechanical.rotational.rotational\"},{\"id\":\"VN\",\"label\":\"VN\",\"type\":\"input\"}],\"Right\":[{\"id\":\"B\",\"label\":\"B\",\"type\":\"foundation.gas.gas\"},{\"id\":\"C\",\"label\":\"C\",\"type\":\"foundation.mechanical.rotational.rotational\"}],\"Top\":[]}"
  Flow Rate Sensor (G) : fl_lib/Gas/Sensors/Flow Rate Sensor (G)  mass_flow_measure=true  volumetric_flow_measure=false  volumetric_flow_conditions=foundation.enum.volumetric_flow_conditions.actual  p_std=0.101325 MPa  T_std=20 degC  energy_flow_measure=false
      settings: InternalSimscapePortConfiguration="{\"Bottom\":[],\"Left\":[{\"id\":\"A\",\"label\":\"A\",\"type\":\"foundation.gas.gas\"}],\"Right\":[{\"id\":\"B\",\"label\":\"B\",\"type\":\"foundation.gas.gas\"},{\"id\":\"M\",\"label\":\"M\",\"type\":\"output\"}],\"Top\":[]}"
  Flow Resistance (G) : fl_lib/Gas/Elements/Flow Resistance (G)  delta_p_nominal=.5 bar  mdot_nominal=.5 kg/s  rho_nominal=1.293 kg/m^3  area=.002 m^2  laminar_fraction=25e-3
      settings: InternalSimscapePortConfiguration="{\"Bottom\":[],\"Left\":[{\"id\":\"A\",\"label\":\"A\",\"type\":\"foundation.gas.gas\"}],\"Right\":[{\"id\":\"B\",\"label\":\"B\",\"type\":\"foundation.gas.gas\"}],\"Top\":[]}"
  Flow Resistance (TL)2 : fl_lib/Thermal Liquid/Elements/Flow Resistance (TL)  delta_p_nominal=0.001 MPa  mdot_nominal=1 kg/s  area=.002 m^2  laminar_fraction=1e-3
  From Spreadsheet1 : FromSpreadsheet  FileName=FCS-heat.xlsx
  Gain : Gain  Gain=max(P64_omega_TLU)*1.546631e-4
  Gain1 : Gain  Gain=.05
  Gain3 : Gain  Gain=max(P64_omega_TLU)*1.546631e-4
  HX002-Temp : Constant  Value=20
  Heat Source : Scope
  Ideal Rotational Motion Sensor : fl_lib/Mechanical/Mechanical Sensors/Ideal Rotational Motion Sensor  reference=foundation.enum.MeasurementReference.difference  acceleration_port=false  velocity_port=true  position_port=false  wrap_angle=false  offset=0 rad
      settings: InternalSimscapePortConfiguration="{\"Bottom\":[],\"Left\":[{\"id\":\"R\",\"label\":\"R\",\"type\":\"foundation.mechanical.rotational.rotational\"}],\"Right\":[{\"id\":\"C\",\"label\":\"C\",\"type\":\"foundation.mechanical.rotational.rotational\"},{\"id\":\"W\",\"label\":\"W\",\"type\":\"output\"}],\"Top\":[]}"
  Ideal Rotational Motion Sensor1 : fl_lib/Mechanical/Mechanical Sensors/Ideal Rotational Motion Sensor  reference=foundation.enum.MeasurementReference.difference  acceleration_port=false  velocity_port=true  position_port=false  wrap_angle=false  offset=0 rad
      settings: InternalSimscapePortConfiguration="{\"Bottom\":[],\"Left\":[{\"id\":\"R\",\"label\":\"R\",\"type\":\"foundation.mechanical.rotational.rotational\"}],\"Right\":[{\"id\":\"C\",\"label\":\"C\",\"type\":\"foundation.mechanical.rotational.rotational\"},{\"id\":\"W\",\"label\":\"W\",\"type\":\"output\"}],\"Top\":[]}"
  Ideal Torque Sensor : fl_lib/Mechanical/Mechanical Sensors/Ideal Torque Sensor
  Ideal Torque Sensor1 : fl_lib/Mechanical/Mechanical Sensors/Ideal Torque Sensor
  Inlet : Subsystem
      settings: PortSchema="{\"entries\":[{\"content\":{\"sides\":[{\"content\":{},\"type\":\"ConnectorPlacement.EquallySpacedRectSide\",\"uuid\":\"383c8b90-d22b-483c-be09-d78d9bde0881\"},{\"content\":{\"connectorIds\":[\"RConn1\"],\"side\":\"RIGHT\"},\"type\":\"ConnectorPlacement.EquallySpacedRectSide\",\"uuid\":\"3dc3e004-4331-4c40-8051-329aa9250422\"},{\"content\":{\"side\":\"TOP\"},\"type\":\"ConnectorPlacement.EquallySpacedRectSide\",\"uuid\":\"aff35d8f-ac03-451a-b72e-dc7bd89924e8\"},{\"content\":{\"connectorIds\":[\"RConn2\",\"RConn3\"],\"side\":\"BOTTOM\"},\"type\":\"ConnectorPlacement.EquallySpacedRectSide\",\"uuid\":\"82493911-a5c4-468a-a003-983b92ffd105\"}]},\"type\":\"ConnectorPlacement.EquallySpacedConnector\",\"uuid\":\"d9a1e9aa-22f5-4e42-bf15-8a8ecd9f58f9\"}],\"packageUris\":[\"http://schema.mathworks.com/mf0/Connector/R2020b\"],\"version\":\"1.0\"}"
  Local Restriction (G) : fl_lib/Gas/Elements/Local Restriction (G)  restriction_type=foundation.enum.restriction_type.variable  restriction_area=1e-3 m^2  min_area=1e-10 m^2  max_area=0.005 m^2  area=0.01 m^2  Cd=0.64  B_lam=0.999
      settings: InternalSimscapePortConfiguration="{\"Bottom\":[],\"Left\":[{\"id\":\"A\",\"label\":\"A\",\"type\":\"foundation.gas.gas\"},{\"id\":\"area_in\",\"label\":\"AR\",\"type\":\"input\"}],\"Right\":[{\"id\":\"B\",\"label\":\"B\",\"type\":\"foundation.gas.gas\"}],\"Top\":[]}"
  Max : MinMax  Function=max  Inputs=2
  Max1 : MinMax  Function=max  Inputs=2
  Mechanical Rotational Reference{1..8} (8 alike) : fl_lib/Mechanical/Rotational Elements/Mechanical Rotational Reference
  MixSEnthalpy-V1_B : Scope  NumInputPorts=8
  Mux : Mux  Inputs=8
  Mux1 : Mux  Inputs=8
  Mux10 : Mux  Inputs=3
  Mux{4,6..9,11} (6 alike) : Mux  Inputs=2
  Mux2 : Mux  Inputs=8
  Mux3 : Mux  Inputs=3
  Mux5 : Mux
  Orifice (G) : SimscapeFluids_lib/Gas/Valves & Orifices/Orifice (G)  orifice_type=foundation.enum.constant_variable.constant  orifice_parameterization=fluids.gas.valves_orifices.enum.OrificeParameterization.Area  opening_characteristic=fluids.gas.valves_orifices.enum.OpeningCharacteristics.Linear  Cv_constant=4  Cv_max=4  L_Cv_TLU=0 : 0.2 : 1  Cv_TLU=[1e-06, .8, 1.6, 2.4, 3.2, 4]  xT_Cv=0.7  Kv_constant=3.95  Kv_max=3.6  L_Kv_TLU=0 : 0.2 : 1  Kv_TLU=[1e-06, .72, 1.44, 2.16, 2.88, 3.6]  xT_Kv=0.75  C_constant=12 l/(bar*s)  B_crit_constant=0.3  C_max=12 l/(bar*s)  B_crit_linear=0.3  L_C_TLU=0 : 0.2 : 1  C_TLU=[1e-05, 2.4, 4.8, 7.2, 9.6, 12] l/(bar*s)  B_crit_TLU=0.3 * ones(1, 6)  m=0.5  T_ref_C=293.15 K  rho_ref_C=1.185 kg/m^3  orifice_area_constant=0.0015 m^2  orifice_area_max=1e-4 m^2  L_orifice_area_TLU=0 : 0.2 : 1  orifice_area_TLU=[1e-10, 2e-05, 4e-05, 6e-05, 8e-05, .0001] m^2  Cd=0.6  leakage_fraction=1e-6  smoothing_factor=0.01  B_lam=0.999  area=0.002 m^2
      settings: InternalSimscapePortConfiguration="{\"Bottom\":[],\"Left\":[{\"id\":\"A\",\"label\":\"A\",\"type\":\"foundation.gas.gas\"}],\"Right\":[{\"id\":\"B\",\"label\":\"B\",\"type\":\"foundation.gas.gas\"}],\"Top\":[]}"
  PANKL_P64_1 : SimscapeFluids_lib/Gas/Turbomachinery/Compressor (G)  parameterization=fluids.gas.turbomachinery.enum.CompressorParameterization.Tabulated  NDes=10000 rpm  piDes=7.5  mdotDes=33 kg/s  efficiencyType=fluids.gas.turbomachinery.enum.EfficiencyType.Analytical  efficiencyValue=0.8  etaMax=0.887  etaMin=0.5  mdotMaxEff=30 kg/s  piMaxEff=7  omega_TLU=P64_omega_TLU rpm  beta_TLU=P64_beta_TLU  pr_TLU=P64_pr_TLU  mdot_TLU=P64_mdot_TLU g/s  eta_TLU=P64_eta_TLU  SMFault=simscape.enum.assert.action.none  a=1.5  b=5  k=0.03  c=3  d=4  cCap=15  dCap=1.0  p_reference=0.101325 MPa  T_reference=288.15 K  mechanical_efficiency=0.9  area_A=.005 m^2  area_B=.005 m^2
      settings: InternalSimscapePortConfiguration="{\"Bottom\":[],\"Left\":[{\"id\":\"A\",\"label\":\"A\",\"type\":\"foundation.gas.gas\"},{\"id\":\"C\",\"label\":\"C\",\"type\":\"foundation.mechanical.rotational.rotational\"}],\"Right\":[{\"id\":\"B\",\"label\":\"B\",\"type\":\"foundation.gas.gas\"},{\"id\":\"R\",\"label\":\"R\",\"type\":\"foundation.mechanical.rotational.rotational\"},{\"id\":\"SM\",\"label\":\"SM\",\"type\":\"output\"}],\"Top\":[]}"
  PANKL_P64_2 : SimscapeFluids_lib/Gas/Turbomachinery/Compressor (G)  parameterization=fluids.gas.turbomachinery.enum.CompressorParameterization.Tabulated  NDes=10000 rpm  piDes=7.5  mdotDes=33 kg/s  efficiencyType=fluids.gas.turbomachinery.enum.EfficiencyType.Analytical  efficiencyValue=0.8  etaMax=0.887  etaMin=0.5  mdotMaxEff=30 kg/s  piMaxEff=7  omega_TLU=P64_omega_TLU rpm  beta_TLU=P64_beta_TLU  pr_TLU=P64_pr_TLU  mdot_TLU=P64_mdot_TLU g/s  eta_TLU=P64_eta_TLU  SMFault=simscape.enum.assert.action.none  a=1.5  b=5  k=0.03  c=3  d=4  cCap=15  dCap=1.0  p_reference=0.101325 MPa  T_reference=288.15 K  mechanical_efficiency=0.9  area_A=.005 m^2  area_B=.005 m^2
      settings: InternalSimscapePortConfiguration="{\"Bottom\":[],\"Left\":[{\"id\":\"A\",\"label\":\"A\",\"type\":\"foundation.gas.gas\"},{\"id\":\"C\",\"label\":\"C\",\"type\":\"foundation.mechanical.rotational.rotational\"}],\"Right\":[{\"id\":\"B\",\"label\":\"B\",\"type\":\"foundation.gas.gas\"},{\"id\":\"R\",\"label\":\"R\",\"type\":\"foundation.mechanical.rotational.rotational\"},{\"id\":\"SM\",\"label\":\"SM\",\"type\":\"output\"}],\"Top\":[]}"
  PID Controller : slpidlib/PID Controller  Controller=PID  Form=Parallel  TimeDomain=Continuous-time  UseExternalTs=off  SampleTime=-1  IntegratorMethod=Forward Euler  FilterMethod=Forward Euler  ControllerParametersSource=internal  P=1  I=1  UseKiTs=off  D=0  N=100  UseFilter=on  TunerSelectOption=Transfer Function Based (PID Tuner App)  InitialConditionSource=internal  InitialConditionForIntegrator=0  InitialConditionForFilter=0  DifferentiatorICPrevScaledInput=0  ExternalReset=none  TrackingMode=off  Kt=1  LimitOutput=off  SatLimitsSource=internal  UpperSaturationLimit=inf  LowerSaturationLimit=-inf  LinearizeAsGain=on  AntiWindupMode=none  Kb=1  LimitIntegrator=off  UpperIntegratorSaturationLimit=inf  LowerIntegratorSaturationLimit=-inf  POutMin=[]  POutMax=[]  IOutMin=[]  IOutMax=[]  DOutMin=[]  DOutMax=[]  NOutMin=[]  NOutMax=[]  SumOutMin=[]  SumOutMax=[]  SaturationOutMin=[]  SaturationOutMax=[]  PParamMin=[]  PParamMax=[]  IParamMin=[]  IParamMax=[]  DParamMin=[]  DParamMax=[]  NParamMin=[]  NParamMax=[]  KbParamMin=[]  KbParamMax=[]  KtParamMin=[]  KtParamMax=[]  KbOutMin=[]  KbOutMax=[]  KtOutMin=[]  KtOutMax=[]  IntegratorOutMin=[]  IntegratorOutMax=[]  FilterOutMin=[]  FilterOutMax=[]  SumI1OutMin=[]  SumI1OutMax=[]  SumI2OutMin=[]  SumI2OutMax=[]  SumI3OutMin=[]  SumI3OutMax=[]  SumI4OutMin=[]  SumI4OutMax=[]  SumDOutMin=[]  SumDOutMax=[]  DifferentiatorOutMin=[]  DifferentiatorOutMax=[]  FilterDiffOutCoefMin=[]  FilterDiffOutCoefMax=[]  ReciprocalOutMin=[]  ReciprocalOutMax=[]  SumDenOutMin=[]  SumDenOutMax=[]  SumNumOutMin=[]  SumNumOutMax=[]  DivideOutMin=[]  DivideOutMax=[]  UdiffTsProdOutMin=[]  UdiffTsProdOutMax=[]  NTsProdOutMin=[]  NTsProdOutMax=[]  UintegralTsProdOutMin=[]  UintegralTsProdOutMax=[]  UngainTsProdOutMin=[]  UngainTsProdOutMax=[]  ClampingZeroOutDataTypeStr=Inherit: Inherit via back propagation  ClampingZeroOutMin=[]  ClampingZeroOutMax=[]  FilterDenConstantOutDataTypeStr=Inherit: Inherit via back propagation  FilterDenConstantOutMin=[]  FilterDenConstantOutMax=[]  PCopyOutDataTypeStr=Inherit: Inherit via back propagation  PCopyOutMin=[]  PCopyOutMax=[]  NCopyOutDataTypeStr=Inherit: Inherit via back propagation  NCopyOutMin=[]  NCopyOutMax=[]  IntegratorContinuousStateAttributes=''  IntegratorStateMustResolveToSignalObject=off  IntegratorRTWStateStorageClass=Auto  FilterContinuousStateAttributes=''  FilterStateMustResolveToSignalObject=off  FilterRTWStateStorageClass=Auto  ParallelPVariant=InternalParameters  IdealPVariant=Disabled  IVariant=InternalParameters  DVariant=InternalParameters  IntegratorVariant=Continuous  SatVariant=Disabled  AWVariant=Passthrough  PCopyVariant=Disabled  TRVariant=Disabled  FdbkBlocksVariant=Forward  IdealPFdbkVariant=Disabled  SatFdbkVariant=Disabled  DerivativeFilterVariant=ContFilter  NVariant=InternalParameters  NCopyVariant=Disabled  FilterICVariant=InternalICsFilter  IntegratorICVariant=InternalICs  ExternalResetVariant=Disabled  TRSumVariant=Passthrough  SumFdbkVariant=Disabled  SumVariant=Sum_PID  TsampFilterVariant=InternalTs  TsampNgainVariant=Passthrough  TsampIntegralVariant=Disabled_SignalSpec  ExternalSaturationOutDataTypeStr=Inherit: Same as second input
  PID Controller1 : slpidlib/PID Controller  Controller=PID  Form=Parallel  TimeDomain=Continuous-time  UseExternalTs=off  SampleTime=-1  IntegratorMethod=Forward Euler  FilterMethod=Forward Euler  ControllerParametersSource=internal  P=1  I=1  UseKiTs=off  D=0  N=100  UseFilter=on  TunerSelectOption=Transfer Function Based (PID Tuner App)  InitialConditionSource=internal  InitialConditionForIntegrator=0  InitialConditionForFilter=0  DifferentiatorICPrevScaledInput=0  ExternalReset=none  TrackingMode=off  Kt=1  LimitOutput=off  SatLimitsSource=internal  UpperSaturationLimit=inf  LowerSaturationLimit=-inf  LinearizeAsGain=on  AntiWindupMode=none  Kb=1  LimitIntegrator=off  UpperIntegratorSaturationLimit=inf  LowerIntegratorSaturationLimit=-inf  POutMin=[]  POutMax=[]  IOutMin=[]  IOutMax=[]  DOutMin=[]  DOutMax=[]  NOutMin=[]  NOutMax=[]  SumOutMin=[]  SumOutMax=[]  SaturationOutMin=[]  SaturationOutMax=[]  PParamMin=[]  PParamMax=[]  IParamMin=[]  IParamMax=[]  DParamMin=[]  DParamMax=[]  NParamMin=[]  NParamMax=[]  KbParamMin=[]  KbParamMax=[]  KtParamMin=[]  KtParamMax=[]  KbOutMin=[]  KbOutMax=[]  KtOutMin=[]  KtOutMax=[]  IntegratorOutMin=[]  IntegratorOutMax=[]  FilterOutMin=[]  FilterOutMax=[]  SumI1OutMin=[]  SumI1OutMax=[]  SumI2OutMin=[]  SumI2OutMax=[]  SumI3OutMin=[]  SumI3OutMax=[]  SumI4OutMin=[]  SumI4OutMax=[]  SumDOutMin=[]  SumDOutMax=[]  DifferentiatorOutMin=[]  DifferentiatorOutMax=[]  FilterDiffOutCoefMin=[]  FilterDiffOutCoefMax=[]  ReciprocalOutMin=[]  ReciprocalOutMax=[]  SumDenOutMin=[]  SumDenOutMax=[]  SumNumOutMin=[]  SumNumOutMax=[]  DivideOutMin=[]  DivideOutMax=[]  UdiffTsProdOutMin=[]  UdiffTsProdOutMax=[]  NTsProdOutMin=[]  NTsProdOutMax=[]  UintegralTsProdOutMin=[]  UintegralTsProdOutMax=[]  UngainTsProdOutMin=[]  UngainTsProdOutMax=[]  ClampingZeroOutDataTypeStr=Inherit: Inherit via back propagation  ClampingZeroOutMin=[]  ClampingZeroOutMax=[]  FilterDenConstantOutDataTypeStr=Inherit: Inherit via back propagation  FilterDenConstantOutMin=[]  FilterDenConstantOutMax=[]  PCopyOutDataTypeStr=Inherit: Inherit via back propagation  PCopyOutMin=[]  PCopyOutMax=[]  NCopyOutDataTypeStr=Inherit: Inherit via back propagation  NCopyOutMin=[]  NCopyOutMax=[]  IntegratorContinuousStateAttributes=''  IntegratorStateMustResolveToSignalObject=off  IntegratorRTWStateStorageClass=Auto  FilterContinuousStateAttributes=''  FilterStateMustResolveToSignalObject=off  FilterRTWStateStorageClass=Auto  ParallelPVariant=InternalParameters  IdealPVariant=Disabled  IVariant=InternalParameters  DVariant=InternalParameters  IntegratorVariant=Continuous  SatVariant=Disabled  AWVariant=Passthrough  PCopyVariant=Disabled  TRVariant=Disabled  FdbkBlocksVariant=Forward  IdealPFdbkVariant=Disabled  SatFdbkVariant=Disabled  DerivativeFilterVariant=ContFilter  NVariant=InternalParameters  NCopyVariant=Disabled  FilterICVariant=InternalICsFilter  IntegratorICVariant=InternalICs  ExternalResetVariant=Disabled  TRSumVariant=Passthrough  SumFdbkVariant=Disabled  SumVariant=Sum_PID  TsampFilterVariant=InternalTs  TsampNgainVariant=Passthrough  TsampIntegralVariant=Disabled_SignalSpec  ExternalSaturationOutDataTypeStr=Inherit: Same as second input
  PS Constant : fl_lib/Physical Signals/Sources/PS Constant  constant=2*pi
  PS Constant1 : fl_lib/Physical Signals/Sources/PS Constant  constant=1
  PS Constant2 : fl_lib/Physical Signals/Sources/PS Constant  constant=2*pi
  PS Product{,1..5} (6 alike) : fl_lib/Physical Signals/Functions/PS Product
  Perfect Insulator : fl_lib/Thermal/Thermal Elements/Perfect Insulator  T_specify=off  T_priority=None  T=293.15 K  T_nominal_specify=off  T_nominal_unit=K  T_nominal_value=1
  Perfect Insulator2 : fl_lib/Thermal/Thermal Elements/Perfect Insulator  T_specify=off  T_priority=None  T=293.15 K  T_nominal_specify=off  T_nominal_unit=K  T_nominal_value=1
  Performance1 : Scope  NumInputPorts=4
  Pipe (G) : fl_lib/Gas/Elements/Pipe (G)  length=1 m  area=0.002 m^2  Dh=0.1 m  length_add=.1 m  roughness=15e-6 m  Re_lam=2000  Re_tur=8000  shape_factor=64  Nu_lam=3.66  p_I_specify=off  p_I_priority=High  p_I=0.101325 MPa  p_I_nominal_specify=off  p_I_nominal_unit=MPa  p_I_nominal_value=1  T_I_specify=off  T_I_priority=High  T_I=293.15 K  T_I_nominal_specify=off  T_I_nominal_unit=K  T_I_nominal_value=1  rho_I_specify=off  rho_I_priority=None  rho_I=1.2 kg/m^3  rho_I_nominal_specify=off  rho_I_nominal_unit=kg/m^3  rho_I_nominal_value=1
  Pipe (G)1 : fl_lib/Gas/Elements/Pipe (G)  length=1 m  area=1 m^2  Dh=0.1 m  length_add=1 m  roughness=15e-6 m  Re_lam=2000  Re_tur=4000  shape_factor=64  Nu_lam=3.66  p_I_specify=off  p_I_priority=High  p_I=0.101325 MPa  p_I_nominal_specify=off  p_I_nominal_unit=MPa  p_I_nominal_value=1  T_I_specify=off  T_I_priority=High  T_I=293.15 K  T_I_nominal_specify=off  T_I_nominal_unit=K  T_I_nominal_value=1  rho_I_specify=off  rho_I_priority=None  rho_I=1.2 kg/m^3  rho_I_nominal_specify=off  rho_I_nominal_unit=kg/m^3  rho_I_nominal_value=1
      settings: LogSimulationData=on
  Pipe (G)2 : fl_lib/Gas/Elements/Pipe (G)  length=1 m  area=1 m^2  Dh=0.1 m  length_add=1 m  roughness=15e-4 m  Re_lam=2000  Re_tur=4000  shape_factor=64  Nu_lam=3.66  p_I_specify=off  p_I_priority=High  p_I=0.101325 MPa  p_I_nominal_specify=off  p_I_nominal_unit=MPa  p_I_nominal_value=1  T_I_specify=off  T_I_priority=High  T_I=293.15 K  T_I_nominal_specify=off  T_I_nominal_unit=K  T_I_nominal_value=1  rho_I_specify=off  rho_I_priority=None  rho_I=1.2 kg/m^3  rho_I_nominal_specify=off  rho_I_nominal_unit=kg/m^3  rho_I_nominal_value=1
  Pipe (G)3 : fl_lib/Gas/Elements/Pipe (G)  length=1 m  area=0.01 m^2  Dh=0.1 m  length_add=1 m  roughness=15e-6 m  Re_lam=2000  Re_tur=4000  shape_factor=64  Nu_lam=3.66  p_I_specify=on  p_I_priority=High  p_I=0.101325 MPa  p_I_nominal_specify=off  p_I_nominal_unit=MPa  p_I_nominal_value=1  T_I_specify=on  T_I_priority=High  T_I=293.15 K  T_I_nominal_specify=off  T_I_nominal_unit=K  T_I_nominal_value=1  rho_I_specify=off  rho_I_priority=None  rho_I=1.2 kg/m^3  rho_I_nominal_specify=off  rho_I_nominal_unit=kg/m^3  rho_I_nominal_value=1
  Pipe (G)4 : fl_lib/Gas/Elements/Pipe (G)  length=1 m  area=0.01 m^2  Dh=0.1 m  length_add=1 m  roughness=15e-6 m  Re_lam=2000  Re_tur=4000  shape_factor=64  Nu_lam=3.66  p_I_specify=on  p_I_priority=High  p_I=0.101325 MPa  p_I_nominal_specify=off  p_I_nominal_unit=MPa  p_I_nominal_value=1  T_I_specify=on  T_I_priority=High  T_I=293.15 K  T_I_nominal_specify=off  T_I_nominal_unit=K  T_I_nominal_value=1  rho_I_specify=off  rho_I_priority=None  rho_I=1.2 kg/m^3  rho_I_nominal_specify=off  rho_I_nominal_unit=kg/m^3  rho_I_nominal_value=1
  Pipe (TL)2 : fl_lib/Thermal Liquid/Elements/Pipe (TL)  length=.2 m  area=0.002 m^2  Dh=0.01 m  length_add=1 m  roughness=15e-6 m  Re_lam=2000  Re_tur=4000  shape_factor=64  Nu_lam=5  dynamic_compressibility=simscape.enum.onoff.on  inertia=simscape.enum.onoff.off  p0=0.101325 MPa  T0=293.15 K  mdot0=0 kg/s
  Plus : Sum  Inputs=+-
  Plus1 : Sum  Inputs=-+
  Power : Scope  NumInputPorts=4
  Pressure Ratio Goal : Product  Inputs=**
  Pressure Ratio Goal1 : Product  Inputs=**
  Pressure 2 OrificeArea : fl_lib/Physical Signals/Functions/PS Gain  gain=0.005 m^2
  Pump Control2 : Subsystem
  Pump2 : fl_lib/Thermal Liquid/Sources/Controlled Mass Flow Rate Source (TL)  power_spec=foundation.enum.power_spec.isentropic  area=.002 m^2
      settings: InternalSimscapePortConfiguration="{\"Bottom\":[],\"Left\":[{\"id\":\"A\",\"label\":\"A\",\"type\":\"foundation.thermal_liquid.thermal_liquid\"},{\"id\":\"M\",\"label\":\"M\",\"type\":\"input\"}],\"Right\":[{\"id\":\"B\",\"label\":\"B\",\"type\":\"foundation.thermal_liquid.thermal_liquid\"}],\"Top\":[]}"
  Radiator2 : fl_lib/Thermal Liquid/Elements/Pipe (TL)  length=1 m  area=.0009375 m^2  Dh=.0028 m  length_add=2.5 m  roughness=15e-6 m  Re_lam=2000  Re_tur=4000  shape_factor=64  Nu_lam=3.66  dynamic_compressibility=simscape.enum.onoff.on  inertia=simscape.enum.onoff.off  p0=.103 MPa  T0=20 degC  mdot0=0 kg/s
  Rotational Electromechanical Converter : fl_lib/Electrical/Electrical Elements/Rotational Electromechanical Converter  K=1.546631e-4 V/rpm  i_specify=off  i_priority=None  i=0 A  i_nominal_specify=off  i_nominal_unit=A  i_nominal_value=1  v_specify=on  v_priority=None  v=24 V  v_nominal_specify=off  v_nominal_unit=V  v_nominal_value=1  t_specify=off  t_priority=None  t=0 N*m  t_nominal_specify=off  t_nominal_unit=N*m  t_nominal_value=1  w_specify=off  w_priority=None  w=0 rad/s  w_nominal_specify=off  w_nominal_unit=rad/s  w_nominal_value=1
  Rotational Electromechanical Converter1 : fl_lib/Electrical/Electrical Elements/Rotational Electromechanical Converter  K=1.546631e-4 V/rpm  i_specify=off  i_priority=None  i=0 A  i_nominal_specify=off  i_nominal_unit=A  i_nominal_value=1  v_specify=on  v_priority=None  v=24 V  v_nominal_specify=off  v_nominal_unit=V  v_nominal_value=1  t_specify=off  t_priority=None  t=0 N*m  t_nominal_specify=off  t_nominal_unit=N*m  t_nominal_value=1  w_specify=off  w_priority=None  w=0 rad/s  w_nominal_specify=off  w_nominal_unit=rad/s  w_nominal_value=1
  S0 : Subsystem
      settings: PortSchema="{\"entries\":[{\"content\":{\"sides\":[{\"content\":{\"connectorIds\":[\"LConn1\"]},\"type\":\"ConnectorPlacement.EquallySpacedRectSide\",\"uuid\":\"872c3fc9-10e2-440a-866c-17ec3b229dcc\"},{\"content\":{\"connectorIds\":[\"RConn1\"],\"side\":\"RIGHT\"},\"type\":\"ConnectorPlacement.EquallySpacedRectSide\",\"uuid\":\"5792e744-d6fd-4953-8a6b-3bc8a25af09f\"},{\"content\":{\"connectorIds\":[\"Out1\"],\"side\":\"TOP\"},\"type\":\"ConnectorPlacement.EquallySpacedRectSide\",\"uuid\":\"2a1362d0-5fde-44c4-8ae5-faebfba0e935\"}]},\"type\":\"ConnectorPlacement.EquallySpacedConnector\",\"uuid\":\"2555ecf8-f6a2-49b2-8cff-d299990cd611\"}],\"packageUris\":[\"http://schema.mathworks.com/mf0/Connector/R2020b\"],\"version\":\"1.0\"}"
  S0_1 : Subsystem
      settings: PortSchema="{\"entries\":[{\"content\":{\"sides\":[{\"content\":{\"connectorIds\":[\"LConn1\"]},\"type\":\"ConnectorPlacement.EquallySpacedRectSide\",\"uuid\":\"872c3fc9-10e2-440a-866c-17ec3b229dcc\"},{\"content\":{\"connectorIds\":[\"RConn1\"],\"side\":\"RIGHT\"},\"type\":\"ConnectorPlacement.EquallySpacedRectSide\",\"uuid\":\"5792e744-d6fd-4953-8a6b-3bc8a25af09f\"},{\"content\":{\"connectorIds\":[\"Out1\"],\"side\":\"TOP\"},\"type\":\"ConnectorPlacement.EquallySpacedRectSide\",\"uuid\":\"2a1362d0-5fde-44c4-8ae5-faebfba0e935\"}]},\"type\":\"ConnectorPlacement.EquallySpacedConnector\",\"uuid\":\"2555ecf8-f6a2-49b2-8cff-d299990cd611\"}],\"packageUris\":[\"http://schema.mathworks.com/mf0/Connector/R2020b\"],\"version\":\"1.0\"}"
  S1 : Subsystem
      settings: PortSchema="{\"entries\":[{\"content\":{\"sides\":[{\"content\":{\"connectorIds\":[\"LConn1\"]},\"type\":\"ConnectorPlacement.EquallySpacedRectSide\",\"uuid\":\"872c3fc9-10e2-440a-866c-17ec3b229dcc\"},{\"content\":{\"connectorIds\":[\"RConn1\"],\"side\":\"RIGHT\"},\"type\":\"ConnectorPlacement.EquallySpacedRectSide\",\"uuid\":\"5792e744-d6fd-4953-8a6b-3bc8a25af09f\"},{\"content\":{\"connectorIds\":[\"Out1\"],\"side\":\"TOP\"},\"type\":\"ConnectorPlacement.EquallySpacedRectSide\",\"uuid\":\"2a1362d0-5fde-44c4-8ae5-faebfba0e935\"}]},\"type\":\"ConnectorPlacement.EquallySpacedConnector\",\"uuid\":\"2555ecf8-f6a2-49b2-8cff-d299990cd611\"}],\"packageUris\":[\"http://schema.mathworks.com/mf0/Connector/R2020b\"],\"version\":\"1.0\"}"
  S2 : Subsystem
      settings: PortSchema="{\"entries\":[{\"content\":{\"sides\":[{\"content\":{\"connectorIds\":[\"LConn1\"]},\"type\":\"ConnectorPlacement.EquallySpacedRectSide\",\"uuid\":\"872c3fc9-10e2-440a-866c-17ec3b229dcc\"},{\"content\":{\"connectorIds\":[\"RConn1\"],\"side\":\"RIGHT\"},\"type\":\"ConnectorPlacement.EquallySpacedRectSide\",\"uuid\":\"5792e744-d6fd-4953-8a6b-3bc8a25af09f\"},{\"content\":{\"connectorIds\":[\"Out1\"],\"side\":\"TOP\"},\"type\":\"ConnectorPlacement.EquallySpacedRectSide\",\"uuid\":\"2a1362d0-5fde-44c4-8ae5-faebfba0e935\"}]},\"type\":\"ConnectorPlacement.EquallySpacedConnector\",\"uuid\":\"2555ecf8-f6a2-49b2-8cff-d299990cd611\"}],\"packageUris\":[\"http://schema.mathworks.com/mf0/Connector/R2020b\"],\"version\":\"1.0\"}"
  S3 : Subsystem
      settings: PortSchema="{\"entries\":[{\"content\":{\"sides\":[{\"content\":{\"connectorIds\":[\"LConn1\"]},\"type\":\"ConnectorPlacement.EquallySpacedRectSide\",\"uuid\":\"872c3fc9-10e2-440a-866c-17ec3b229dcc\"},{\"content\":{\"connectorIds\":[\"RConn1\"],\"side\":\"RIGHT\"},\"type\":\"ConnectorPlacement.EquallySpacedRectSide\",\"uuid\":\"5792e744-d6fd-4953-8a6b-3bc8a25af09f\"},{\"content\":{\"connectorIds\":[\"Out1\"],\"side\":\"TOP\"},\"type\":\"ConnectorPlacement.EquallySpacedRectSide\",\"uuid\":\"2a1362d0-5fde-44c4-8ae5-faebfba0e935\"}]},\"type\":\"ConnectorPlacement.EquallySpacedConnector\",\"uuid\":\"2555ecf8-f6a2-49b2-8cff-d299990cd611\"}],\"packageUris\":[\"http://schema.mathworks.com/mf0/Connector/R2020b\"],\"version\":\"1.0\"}"
  S5 : Subsystem
      settings: PortSchema="{\"entries\":[{\"content\":{\"sides\":[{\"content\":{\"connectorIds\":[\"LConn1\"]},\"type\":\"ConnectorPlacement.EquallySpacedRectSide\",\"uuid\":\"872c3fc9-10e2-440a-866c-17ec3b229dcc\"},{\"content\":{\"connectorIds\":[\"RConn1\"],\"side\":\"RIGHT\"},\"type\":\"ConnectorPlacement.EquallySpacedRectSide\",\"uuid\":\"5792e744-d6fd-4953-8a6b-3bc8a25af09f\"},{\"content\":{\"connectorIds\":[\"Out1\"],\"side\":\"TOP\"},\"type\":\"ConnectorPlacement.EquallySpacedRectSide\",\"uuid\":\"2a1362d0-5fde-44c4-8ae5-faebfba0e935\"}]},\"type\":\"ConnectorPlacement.EquallySpacedConnector\",\"uuid\":\"2555ecf8-f6a2-49b2-8cff-d299990cd611\"}],\"packageUris\":[\"http://schema.mathworks.com/mf0/Connector/R2020b\"],\"version\":\"1.0\"}"
  S7 : Subsystem
      settings: PortSchema="{\"entries\":[{\"content\":{\"sides\":[{\"content\":{\"connectorIds\":[\"LConn1\"]},\"type\":\"ConnectorPlacement.EquallySpacedRectSide\",\"uuid\":\"872c3fc9-10e2-440a-866c-17ec3b229dcc\"},{\"content\":{\"connectorIds\":[\"RConn1\"],\"side\":\"RIGHT\"},\"type\":\"ConnectorPlacement.EquallySpacedRectSide\",\"uuid\":\"5792e744-d6fd-4953-8a6b-3bc8a25af09f\"},{\"content\":{\"connectorIds\":[\"Out1\"],\"side\":\"TOP\"},\"type\":\"ConnectorPlacement.EquallySpacedRectSide\",\"uuid\":\"2a1362d0-5fde-44c4-8ae5-faebfba0e935\"}]},\"type\":\"ConnectorPlacement.EquallySpacedConnector\",\"uuid\":\"2555ecf8-f6a2-49b2-8cff-d299990cd611\"}],\"packageUris\":[\"http://schema.mathworks.com/mf0/Connector/R2020b\"],\"version\":\"1.0\"}"
  S8 : Subsystem
      settings: PortSchema="{\"entries\":[{\"content\":{\"sides\":[{\"content\":{\"connectorIds\":[\"LConn1\"]},\"type\":\"ConnectorPlacement.EquallySpacedRectSide\",\"uuid\":\"872c3fc9-10e2-440a-866c-17ec3b229dcc\"},{\"content\":{\"connectorIds\":[\"RConn1\"],\"side\":\"RIGHT\"},\"type\":\"ConnectorPlacement.EquallySpacedRectSide\",\"uuid\":\"5792e744-d6fd-4953-8a6b-3bc8a25af09f\"},{\"content\":{\"connectorIds\":[\"Out1\"],\"side\":\"TOP\"},\"type\":\"ConnectorPlacement.EquallySpacedRectSide\",\"uuid\":\"2a1362d0-5fde-44c4-8ae5-faebfba0e935\"}]},\"type\":\"ConnectorPlacement.EquallySpacedConnector\",\"uuid\":\"2555ecf8-f6a2-49b2-8cff-d299990cd611\"}],\"packageUris\":[\"http://schema.mathworks.com/mf0/Connector/R2020b\"],\"version\":\"1.0\"}"
  SEntropy-V1_B : Scope  NumInputPorts=8
  SHeat-V1_B : Scope  NumInputPorts=8
  Simulink-PS Converter1 : nesl_utility/Simulink-PS Converter  PhysicalDomain=network_engine_domain  SubClassName=ps_input  LeftPortType=input  RightPortType=output  PseudoPeriodic=off  Frequencies=[]  NoiseDistribution=none  NoiseParameters=[]  Unit=kW  AffineConversion=off  FilteringAndDerivatives=provide  SimscapeFilterOrder=1  InputFilterTimeConstant=0.001  UdotUserProvided=0
  Simulink-PS Converter2 : nesl_utility/Simulink-PS Converter  PhysicalDomain=network_engine_domain  SubClassName=ps_input  LeftPortType=input  RightPortType=output  PseudoPeriodic=off  Frequencies=[]  NoiseDistribution=none  NoiseParameters=[]  Unit=1  AffineConversion=off  FilteringAndDerivatives=filter  SimscapeFilterOrder=1  InputFilterTimeConstant=0.005  UdotUserProvided=0
  Simulink-PS Converter4 : nesl_utility/Simulink-PS Converter  PhysicalDomain=network_engine_domain  SubClassName=ps_input  LeftPortType=input  RightPortType=output  PseudoPeriodic=off  Frequencies=[]  NoiseDistribution=none  NoiseParameters=[]  Unit=1  AffineConversion=off  FilteringAndDerivatives=filter  SimscapeFilterOrder=1  InputFilterTimeConstant=0.005  UdotUserProvided=0
  Simulink-PS Converter6 : nesl_utility/Simulink-PS Converter  PhysicalDomain=network_engine_domain  SubClassName=ps_input  LeftPortType=input  RightPortType=output  PseudoPeriodic=off  Frequencies=[]  NoiseDistribution=none  NoiseParameters=[]  Unit=1  AffineConversion=off  FilteringAndDerivatives=provide  SimscapeFilterOrder=1  InputFilterTimeConstant=0.001  UdotUserProvided=0
  Subsystem3 : Subsystem
  Switch2 : Switch  Criteria=u2 > Threshold  Threshold=1.4  SaturateOnIntegerOverflow=off  InputSameDT=off
  Switch3 : Switch  Criteria=u2 > Threshold  Threshold=1.4  SaturateOnIntegerOverflow=off  InputSameDT=off
  Switch4 : Switch  Criteria=u2 > Threshold  Threshold=1.4  SaturateOnIntegerOverflow=off  InputSameDT=off
  Thermal Mass : fl_lib/Thermal/Thermal Elements/Thermal Mass  mass_type=foundation.enum.constant_variable.constant  mass=1000 kg  sp_heat=447 J/(K*kg)  mass_min=1e-6 kg  num_ports=foundation.enum.numPorts2.one  m_specify=off  m_priority=High  m=1 kg  m_nominal_specify=off  m_nominal_unit=kg  m_nominal_value=1  T_specify=off  T_priority=High  T=300 K  T_nominal_specify=off  T_nominal_unit=K  T_nominal_value=1  Q_specify=off  Q_priority=None  Q=0 W  Q_nominal_specify=off  Q_nominal_unit=W  Q_nominal_value=1
  Thermal Mass1 : fl_lib/Thermal/Thermal Elements/Thermal Mass  mass_type=foundation.enum.constant_variable.constant  mass=1000 kg  sp_heat=447 J/(K*kg)  mass_min=1e-6 kg  num_ports=foundation.enum.numPorts2.one  m_specify=off  m_priority=High  m=1 kg  m_nominal_specify=off  m_nominal_unit=kg  m_nominal_value=1  T_specify=off  T_priority=High  T=300 K  T_nominal_specify=off  T_nominal_unit=K  T_nominal_value=1  Q_specify=off  Q_priority=None  Q=0 W  Q_nominal_specify=off  Q_nominal_unit=W  Q_nominal_value=1
  Thermal Mass3 : fl_lib/Thermal/Thermal Elements/Thermal Mass  mass_type=foundation.enum.constant_variable.constant  mass=1 kg  sp_heat=910 J/kg/K  mass_min=1e-6 kg  num_ports=foundation.enum.numPorts2.one  m_specify=off  m_priority=High  m=1 kg  m_nominal_specify=off  m_nominal_unit=kg  m_nominal_value=1  T_specify=on  T_priority=High  T=20 degC  T_nominal_specify=off  T_nominal_unit=K  T_nominal_value=1  Q_specify=off  Q_priority=None  Q=0 W  Q_nominal_specify=off  Q_nominal_unit=W  Q_nominal_value=1
  Thermal Mass4 : fl_lib/Thermal/Thermal Elements/Thermal Mass  mass_type=foundation.enum.constant_variable.constant  mass=10 kg  sp_heat=447 J/(K*kg)  mass_min=1e-6 kg  num_ports=foundation.enum.numPorts2.one  m_specify=off  m_priority=High  m=1 kg  m_nominal_specify=off  m_nominal_unit=kg  m_nominal_value=1  T_specify=off  T_priority=High  T=300 K  T_nominal_specify=off  T_nominal_unit=K  T_nominal_value=1  Q_specify=off  Q_priority=None  Q=0 W  Q_nominal_specify=off  Q_nominal_unit=W  Q_nominal_value=1
  Thermal Reference : fl_lib/Thermal/Thermal Elements/Thermal Reference
  Transfer Fcn : TransferFcn  Denominator=[2 1]
  Transfer Fcn1 : TransferFcn  Denominator=[2 1]
  Voltage Sensor : fl_lib/Electrical/Electrical Sensors/Voltage Sensor
  Voltage Sensor1 : fl_lib/Electrical/Electrical Sensors/Voltage Sensor
  XY Graph : Record  FileSettingsInternal="{\"entries\":[{\"content\":{\"excelSettings\":{\"content\":{},\"type\":\"Streamout.ExcelSettings\"}},\"type\":\"Streamout.FileSettingStorage\",\"uuid\":\"9b20f94d-8001-4f72-994a-3fb3a226c2c1\"}],\"packageUris\":[\"http://schema.mathworks.com/mf0/streamout_blocks/R2020a\"],\"version\":\"1.0\"}"  Layout=[1 1]  SignalsInternal="{\"entries\":[{\"content\":{\"signals\":[{\"content\":{\"blockPath\":[\"H175_PANKL_V1a/XY Graph\"],\"dimensions\":[1,1],\"domain\":\"H175_PANKL_V1a/XY Graph\",\"lineColor\":\"#a2142f\",\"plots\":[1],\"port\":1,\"sid\":[\"\"],\"signalID\":10105,\"signalName\":\"Subsystem3:19\"},\"type\":\"RecordBlkView.Signal\",\"uuid\":\"3fba7e24-6059-4eb0-ba5e-120f9d6b7f9f\"},{\"content\":{\"blockPath\":[\"H175_PANKL_V1a/XY Graph\"],\"dimensions\":[1,1],\"domain\":\"H175_PANKL_V1a/XY Graph\",\"lineColor\":\"#139fff\",\"plots\":[1],\"port\":2,\"sid\":[\"\"],\"signalID\":10109,\"signalName\":\"Divide\"},\"type\":\"RecordBlkView.Signal\",\"uuid\":\"d57a0b9d-e476-48e4-8a6c-3b89d4a77c6b\"}]},\"type\":\"RecordBlkView.InputSignals\",\"uuid\":\"13d39f8b-fc2a-4c25-ace1-a3bf3046e0f7\"}],\"packageUris\":[\"http://schema.mathworks.com/mf0/streamout_blocks/R2020a\"],\"version\":\"1.0\"}"  VisualizationBindings="{\"xyplotplugin\":{\"info\":[{\"series\":[],\"subplotID\":1}]}}"  CompatibilityTag=XY
  XY Graph1 : Record  FileSettingsInternal="{\"entries\":[{\"content\":{\"excelSettings\":{\"content\":{},\"type\":\"Streamout.ExcelSettings\"}},\"type\":\"Streamout.FileSettingStorage\",\"uuid\":\"0c60d94a-d59d-48c1-ad2e-f9d1eec8d216\"}],\"packageUris\":[\"http://schema.mathworks.com/mf0/streamout_blocks/R2020a\"],\"version\":\"1.0\"}"  Layout=[1 1]  SignalsInternal="{\"entries\":[{\"content\":{\"signals\":[{\"content\":{\"blockPath\":[\"H175_PANKL_V1a/XY Graph1\"],\"dimensions\":[1,1],\"domain\":\"H175_PANKL_V1a/XY Graph1\",\"lineColor\":\"#fe330a\",\"port\":1,\"sid\":[\"\"],\"signalID\":10113,\"signalName\":\"Subsystem3:19\"},\"type\":\"RecordBlkView.Signal\",\"uuid\":\"f9263a01-77ca-4694-b583-6fdae6d0aeaa\"},{\"content\":{\"blockPath\":[\"H175_PANKL_V1a/XY Graph1\"],\"dimensions\":[1,1],\"domain\":\"H175_PANKL_V1a/XY Graph1\",\"lineColor\":\"#22b573\",\"port\":2,\"sid\":[\"\"],\"signalID\":10117,\"signalName\":\"Divide1\"},\"type\":\"RecordBlkView.Signal\",\"uuid\":\"6cc41745-e698-4e7e-b97f-04599ad5397b\"}]},\"type\":\"RecordBlkView.InputSignals\",\"uuid\":\"79a2bd46-73be-437b-bc01-6db795643d38\"}],\"packageUris\":[\"http://schema.mathworks.com/mf0/streamout_blocks/R2020a\"],\"version\":\"1.0\"}"  VisualizationBindings="{\"xyplotplugin\":{\"info\":[{\"series\":[],\"subplotID\":1}]}}"  CompatibilityTag=XY
  a : SimscapeFluids_lib/Gas/Turbomachinery/Compressor (G)  parameterization=fluids.gas.turbomachinery.enum.CompressorParameterization.Tabulated  NDes=10000 rpm  piDes=7.5  mdotDes=33 kg/s  efficiencyType=fluids.gas.turbomachinery.enum.EfficiencyType.Analytical  efficiencyValue=0.8  etaMax=0.887  etaMin=0.5  mdotMaxEff=30 kg/s  piMaxEff=7  omega_TLU=P64_omega_TLU rpm  beta_TLU=P64_beta_TLU  pr_TLU=P64_pr_TLU  mdot_TLU=P64_mdot_TLU g/s  eta_TLU=P64_eta_TLU  SMFault=simscape.enum.assert.action.none  a=1.5  b=5  k=0.03  c=3  d=4  cCap=15  dCap=1.0  p_reference=0.101325 MPa  T_reference=288.15 K  mechanical_efficiency=0.9  area_A=.005 m^2  area_B=.005 m^2
      settings: LogSimulationData=on  InternalSimscapePortConfiguration="{\"Bottom\":[],\"Left\":[{\"id\":\"A\",\"label\":\"A\",\"type\":\"foundation.gas.gas\"},{\"id\":\"C\",\"label\":\"C\",\"type\":\"foundation.mechanical.rotational.rotational\"}],\"Right\":[{\"id\":\"B\",\"label\":\"B\",\"type\":\"foundation.gas.gas\"},{\"id\":\"R\",\"label\":\"R\",\"type\":\"foundation.mechanical.rotational.rotational\"},{\"id\":\"SM\",\"label\":\"SM\",\"type\":\"output\"}],\"Top\":[]}"
  mFlow-V1_B : Scope  NumInputPorts=8
  wires:
  S1/1(Out1) -> [S1]
  S2/1(Out1) -> [S2]
  S3/1(Out1) -> [S3]
  S5/1(Out1) -> [S5]
  S7/1(Out1) -> [S7]
  [CMP1_rpm] -> Mux6/1
  S0/1(Out1) -> [S0]
  S0_1/1(Out1) -> [S0_1]
  S8/1(Out1) -> [S8]
  HX002-Temp/1 -> Pump Control2/1(T_set)
  CMP2_SM1/1 -> [CMP2_SM1]
  [CMP1_SM1] -> Mux3/1
  [CMP1_SM2] -> Mux3/2
  [CMP2_SM1] -> Mux3/3
  [CMP2_nM] -> Mux4/1
  CMP2_nM/1 -> [CMP2_nM]
  [CMP2_rpm] -> Mux6/2
  CMP2_rpm/1 -> [CMP2_rpm]
  [S0] -> Subsystem3/1(In1)
  [S0_1] -> Subsystem3/2(In2)
  [S1] -> Subsystem3/3(In3)
  [S2] -> Subsystem3/4(In4)
  [S3] -> Subsystem3/5(In5)
  [S5] -> Subsystem3/6(In6)
  [S7] -> Subsystem3/7(In7)
  [S8] -> Subsystem3/8(In8)
  Subsystem3/1(<aPres_S0>) -> Mux/1, Divide1/2, Divide/2
  Subsystem3/2(<aPres_S0_1>) -> Mux/2
  Subsystem3/3(<aPres_S1>) -> Mux/3, Divide/1
  Subsystem3/4(<aPres_S2>) -> Mux/4
  Subsystem3/5(<aPres_S3>) -> Divide1/1, Mux/5
  Subsystem3/6(<aPres_S5>) -> Mux/6
  Subsystem3/7(<aPres_S7>) -> Mux/7
  Subsystem3/8(<aPres_S8>) -> Mux/8
  Subsystem3/9(<aTemp_S0>) -> Mux1/1
  Subsystem3/10(<aTemp_S0_1>) -> Mux1/2
  Subsystem3/11(<aTemp_S1>) -> Mux1/3
  Subsystem3/12(<aTemp_S2>) -> Mux1/4
  Subsystem3/13(<aTemp_S3>) -> Mux1/5
  Subsystem3/14(<aTemp_S5>) -> Mux1/6
  Subsystem3/15(<aTemp_S7>) -> Mux1/7
  Subsystem3/16(<aTemp_S8>) -> Mux1/8
  Subsystem3/17(<mFlow_S0>) -> mFlow-V1_B/1
  Subsystem3/18(<mFlow_S0_1>) -> mFlow-V1_B/2
  Subsystem3/19(<mFlow_S1>) -> Mux7/1, XY Graph1/1, XY Graph/1, mFlow-V1_B/3
  Subsystem3/20(<mFlow_S2>) -> mFlow-V1_B/4
  Subsystem3/21(<mFlow_S3>) -> mFlow-V1_B/5
  Subsystem3/22(<mFlow_S5>) -> mFlow-V1_B/6
  Subsystem3/23(<mFlow_S7>) -> mFlow-V1_B/7
  Subsystem3/24(<mFlow_S8>) -> mFlow-V1_B/8
  Subsystem3/25(<MixSEnthalpy_S0>) -> MixSEnthalpy-V1_B/1
  Subsystem3/26(<MixSEnthalpy_S0_1>) -> MixSEnthalpy-V1_B/2
  Subsystem3/27(<MixSEnthalpy_S1>) -> MixSEnthalpy-V1_B/3
  Subsystem3/28(<MixSEnthalpy_S2>) -> MixSEnthalpy-V1_B/4
  Subsystem3/29(<MixSEnthalpy_S3>) -> MixSEnthalpy-V1_B/5
  Subsystem3/30(<MixSEnthalpy_S5>) -> MixSEnthalpy-V1_B/6
  Subsystem3/31(<MixSEnthalpy_S7>) -> MixSEnthalpy-V1_B/7
  Subsystem3/32(<MixSEnthalpy_S8>) -> MixSEnthalpy-V1_B/8
  Subsystem3/33(<MixDensity_S0>) -> Mux2/1
  Subsystem3/34(<MixDensity_S0_1>) -> Mux2/2
  Subsystem3/35(<MixDensity_S1>) -> Mux2/3
  Subsystem3/36(<MixDensity_S2>) -> Mux2/4
  Subsystem3/37(<MixDensity_S3>) -> Mux2/5
  Subsystem3/38(<MixDensity_S5>) -> Mux2/6
  Subsystem3/39(<MixDensity_S7>) -> Mux2/7
  Subsystem3/40(<MixDensity_S8>) -> Mux2/8
  Subsystem3/41(<SHeat_S0>) -> SHeat-V1_B/1
  Subsystem3/42(<SHeat_S0_1>) -> SHeat-V1_B/2
  Subsystem3/43(<SHeat_S1>) -> SHeat-V1_B/3
  Subsystem3/44(<SHeat_S2>) -> SHeat-V1_B/4
  Subsystem3/45(<SHeat_S3>) -> SHeat-V1_B/5
  Subsystem3/46(<SHeat_S5>) -> SHeat-V1_B/6
  Subsystem3/47(<SHeat_S7>) -> SHeat-V1_B/7
  Subsystem3/48(<SHeat_S8>) -> SHeat-V1_B/8
  Subsystem3/49(<SEntropy_S0>) -> SEntropy-V1_B/1
  Subsystem3/50(<SEntropy_S0_1>) -> SEntropy-V1_B/2
  Subsystem3/51(<SEntropy_S1>) -> SEntropy-V1_B/3
  Subsystem3/52(<SEntropy_S2>) -> SEntropy-V1_B/4
  Subsystem3/53(<SEntropy_S3>) -> SEntropy-V1_B/5
  Subsystem3/54(<SEntropy_S5>) -> SEntropy-V1_B/6
  Subsystem3/55(<SEntropy_S7>) -> SEntropy-V1_B/7
  Subsystem3/56(<SEntropy_S8>) -> SEntropy-V1_B/8
  [S5] -> Pump Control2/2(In2)
  Gain1/1 -> Simulink-PS Converter1/1
  Divide/1 -> XY Graph/2
  Divide1/1 -> XY Graph1/2
  CMP1_rpm/1 -> [CMP1_rpm]
  CMP1_nM/1 -> [CMP1_nM]
  CMP1_SM1/1 -> [CMP1_SM1]
  CMP1_SM2/1 -> [CMP1_SM2]
  CMP2_eP/1 -> [CMP2_eP]
  CMP1_eP/1 -> [CMP1_eP]
  [CMP2_eP] -> Mux5/4
  [CMP1_eP] -> Mux5/3
  CMP1_nP/1 -> [CMP1_nP]
  CMP2_nP/1 -> [CMP2_nP]
  [CMP1_nP] -> Mux5/1
  [CMP2_nP] -> Mux5/2
  Mux/1 -> Performance1/1
  Mux1/1 -> Performance1/2
  [CMP1_nM] -> Mux4/2
  Mux3/1 -> Power/1
  Mux4/1 -> Power/2
  Mux6/1 -> Power/3
  Mux5/1 -> Power/4
  From Spreadsheet1/1 -> Heat Source/1, Gain1/1
  Mux2/1 -> Performance1/4
  Mux7/1 -> Performance1/3
  CMP1_eP4/1 -> Mux7/2
  Switch3/1 -> Plus/1
  Exp2/1 -> Switch4/2
  Mux9/1 -> Control Signals/1
  Transfer Fcn/1 -> Gain/1
  Switch2/1 -> Pressure Ratio Goal/1
  Constant8/1 -> Switch4/3
  Pressure Ratio Goal/1 -> Mux8/1, Plus/2
  PID Controller/1 -> Transfer Fcn/1, Mux9/1
  Constant9/1 -> Switch4/1
  Exp/1 -> Switch2/2
  Mux8/1 -> Control Signals/2
  Plus/1 -> Mux9/2, PID Controller/1
  Constant2/1 -> Switch2/3
  Constant6/1 -> Pressure Ratio Goal/2
  Exp1/1 -> Switch3/2
  Constant1/1 -> Switch3/3
  Bus Selector/1 -> Switch3/1  "<aPres_S0_1>"
  Switch4/1 -> Simulink-PS Converter6/1
  [S0_1] -> Bus Selector/1
  [S0] -> Bus Selector1/1
  Bus Selector1/1 -> Max1/2, Mux8/2, Exp/1, Switch2/1, Exp1/1  "<aPres_S0>"
  Constant3/1 -> Pressure Ratio Goal1/2
  Plus1/1 -> Mux11/2, PID Controller1/1
  Pressure Ratio Goal1/1 -> Mux10/2, Plus1/2
  PID Controller1/1 -> Mux11/1, Transfer Fcn1/1
  Transfer Fcn1/1 -> Gain3/1
  [S1] -> Bus Selector2/1
  Bus Selector2/1 -> Mux10/3, Pressure Ratio Goal1/1  "<aPres_S1>"
  Mux10/1 -> Control Signals1/2
  Mux11/1 -> Control Signals1/1
  Gain/1 -> Simulink-PS Converter2/1
  Constant5/1 -> Max/1
  Max/1 -> Simulink-PS Converter4/1
  Gain3/1 -> Max/2
  Constant4/1 -> Max1/1
  Max1/1 -> Exp2/1
  Constant/1 -> Mux10/1, Plus1/1
  connections:
  a/RConn3 -- CMP2_SM1/LConn1
  CMP2_rpm/LConn1 -- ./RConn1
  Mechanical Rotational Reference2/LConn1 -- a/LConn2
  S5/RConn1 -- Expander-55mm/LConn1
  PS Constant1/RConn1 -- Expander-55mm/LConn3
  Thermal Reference/LConn1 -- Controlled Heat Flow Rate Source/RConn2
  Pipe (G)/LConn2 -- Thermal Mass4/LConn1 -- Convective Heat Transfer/RConn1
  Simulink-PS Converter1/RConn1 -- Controlled Heat Flow Rate Source/RConn1
  Convective Heat Transfer/LConn1 -- Controlled Heat Flow Rate Source/LConn1
  a/LConn1 -- S1/RConn1
  S2/RConn1 -- Pipe (G)1/LConn1
  a/RConn1 -- Constant Volume Chamber (G)1/LConn1
  Expander-55mm/RConn2 -- Mechanical Rotational Reference3/LConn1
  Inlet/RConn1 -- S0/LConn1
  S0_1/RConn1 -- Pipe (G)2/LConn1
  Convective Heat Transfer7/LConn1 -- Pipe (G)2/LConn2
  Pipe (G)4/LConn1 -- Pipe (G)/RConn1
  S3/RConn1 -- Pipe (G)1/RConn1
  Convective Heat Transfer1/RConn1 -- Pipe (G)3/LConn2
  Coolant Tank2/RConn1 -- Pump2/LConn1 -- Flow Resistance (TL)2/RConn1
  Pipe (TL)2/LConn1 -- Pump2/RConn1 -- Coolant Properties2/RConn1
  Convective Heat Transfer8/LConn1 -- Pipe (G)1/LConn2
  Radiator2/RConn1 -- Flow Resistance (TL)2/LConn1
  Thermal Mass3/LConn1 -- Environment Temperature2/LConn1 -- Convective Heat Transfer5/RConn1
  Radiator2/LConn1 -- Pipe (TL)2/RConn1
  Pipe (G)4/LConn2 -- Convective Heat Transfer2/RConn1
  S7/LConn1 -- Expander-55mm/RConn1
  Constant Volume Chamber (G)/RConn1 -- Local Restriction (G)/RConn1 -- S0_1/LConn1
  Thermal Mass1/LConn1 -- Convective Heat Transfer8/RConn1 -- Pipe (TL)2/LConn2 -- Thermal Mass/LConn1 -- Convective Heat Transfer7/RConn1 -- Convective Heat Transfer1/LConn1 -- Convective Heat Transfer2/LConn1
  Convective Heat Transfer5/LConn1 -- Radiator2/LConn2
  Controlled Reservoir (G)1/LConn1 -- Orifice (G)/RConn1
  S7/RConn1 -- Pipe (G)3/LConn1
  Perfect Insulator/LConn1 -- Constant Volume Chamber (G)/LConn2
  S1/LConn1 -- Pipe (G)2/RConn1
  PANKL_P64_1/RConn1 -- Flow Rate Sensor (G)/RConn1 -- Constant Volume Chamber (G)/LConn1
  Flow Resistance (G)/RConn1 -- Pipe (G)/LConn1
  Flow Resistance (G)/LConn1 -- S3/LConn1
  Mechanical Rotational Reference1/LConn1 -- PANKL_P64_2/LConn2
  Mechanical Rotational Reference4/LConn1 -- PANKL_P64_1/LConn2
  S0/RConn1 -- PANKL_P64_2/LConn1 -- Local Restriction (G)/LConn1 -- PANKL_P64_1/LConn1
  Expander-55mm/LConn2 -- a/RConn2 -- Ideal Torque Sensor/RConn1
  Pump Control2/RConn1 -- Pump2/LConn2
  Perfect Insulator2/LConn1 -- Constant Volume Chamber (G)1/LConn2
  Constant Volume Chamber (G)1/RConn1 -- S2/LConn1
  Rotational Electromechanical Converter/LConn2 -- Ideal Rotational Motion Sensor/LConn1 -- Ideal Torque Sensor/LConn1
  Rotational Electromechanical Converter/RConn1 -- Electrical Reference/LConn1 -- Controlled Voltage Source2/RConn2
  Mechanical Rotational Reference6/LConn1 -- Rotational Electromechanical Converter/RConn2
  ./LConn1 -- Ideal Rotational Motion Sensor/RConn2 -- PS Product4/LConn1
  Mechanical Rotational Reference5/LConn1 -- Ideal Rotational Motion Sensor/RConn1
  .3/RConn1 -- PS Product4/LConn2
  PANKL_P64_1/RConn2 -- Ideal Torque Sensor1/RConn1 -- PANKL_P64_2/RConn2
  Controlled Voltage Source1/RConn2 -- Electrical Reference1/LConn1 -- Rotational Electromechanical Converter1/RConn1
  Ideal Torque Sensor1/RConn2 -- PS Product2/LConn2 -- CMP1_nM/LConn1
  Mechanical Rotational Reference7/LConn1 -- Ideal Rotational Motion Sensor1/RConn1
  .2/LConn1 -- Ideal Rotational Motion Sensor1/RConn2 -- .4/LConn1
  Mechanical Rotational Reference8/LConn1 -- Rotational Electromechanical Converter1/RConn2
  .4/RConn1 -- CMP1_rpm/LConn1
  CMP1_SM1/LConn1 -- PANKL_P64_1/RConn3
  PANKL_P64_2/RConn3 -- CMP1_SM2/LConn1
  Voltage Sensor/LConn1 -- Controlled Voltage Source2/LConn1 -- Current Sensor/LConn1
  Current Sensor/RConn2 -- Rotational Electromechanical Converter/LConn1
  Voltage Sensor/RConn2 -- Electrical Reference2/LConn1
  Current Sensor/RConn1 -- PS Product/LConn1
  Voltage Sensor/RConn1 -- PS Product/LConn2
  PS Product/RConn1 -- CMP2_eP/LConn1
  Voltage Sensor1/LConn1 -- Controlled Voltage Source1/LConn1 -- Current Sensor1/LConn1
  Current Sensor1/RConn1 -- PS Product1/LConn1
  Voltage Sensor1/RConn1 -- PS Product1/LConn2
  PS Product1/RConn1 -- CMP1_eP/LConn1
  Voltage Sensor1/RConn2 -- Electrical Reference3/LConn1
  Current Sensor1/RConn2 -- Rotational Electromechanical Converter1/LConn1
  PS Product2/RConn1 -- PS Product3/LConn1
  PS Product3/LConn2 -- PS Constant/RConn1
  PS Product3/RConn1 -- CMP1_nP/LConn1
  PS Product5/RConn1 -- CMP2_nP/LConn1
  PS Constant2/RConn1 -- PS Product5/LConn2
  PS Product4/RConn1 -- PS Product5/LConn1
  Ideal Torque Sensor1/LConn1 -- Rotational Electromechanical Converter1/LConn2 -- Ideal Rotational Motion Sensor1/LConn1
  .2/RConn1 -- PS Product2/LConn1
  CMP2_nM/LConn1 -- Ideal Torque Sensor/RConn2 -- .3/LConn1
  Orifice (G)/LConn1 -- S8/RConn1
  Controlled Reservoir (G)1/RConn1 -- Inlet/RConn3
  Controlled Reservoir (G)1/RConn2 -- Inlet/RConn2
  S8/LConn1 -- Pipe (G)3/RConn1
  S5/LConn1 -- Pipe (G)4/RConn1
  Simulink-PS Converter4/RConn1 -- Controlled Voltage Source2/RConn1
  PANKL_P64_2/RConn1 -- Flow Rate Sensor (G)/LConn1
  CMP1_eP4/LConn1 -- Flow Rate Sensor (G)/RConn2
  Simulink-PS Converter6/RConn1 -- Pressure 2 OrificeArea/LConn1
  Local Restriction (G)/LConn2 -- Pressure 2 OrificeArea/RConn1
  Simulink-PS Converter2/RConn1 -- Controlled Voltage Source1/RConn1
